simulink model "ForwardKinematic_YuMi"  (R2024a)
(part 9 of 23)

(5148155107303929*sin(q1L))/9007199254740992))/36893488147419103232 + sin(q2L)*((5148155107303929*cos(q1L))/9007199254740992 + (1888752292310023*sin(q1L))/18014398509481984)))/36893488147419103232 + cos(q3L)*((16506520352940097956833727997725*sin(q2L))/20282409603651670423947251286016 - cos(q2L)*((5148155107303929*cos(q1L))/9007199254740992 + (1888752292310023*sin(q1L))/18014398509481984) + (7514214926474921*sin(q2L)*((1888752292310023*cos(q1L))/18014398509481984 - (5148155107303929*sin(q1L))/9007199254740992))/36893488147419103232)))/332306998946228968225951765070086144 + (508577317689771495245073589786522929324694383585*sin(q3L)*((16506520352940097956833727997725*cos(q2L))/20282409603651670423947251286016 + (7514214926474921*cos(q2L)*((1888752292310023*cos(q1L))/18014398509481984 - (5148155107303929*sin(q1L))/9007199254740992))/36893488147419103232 + sin(q2L)*((5148155107303929*cos(q1L))/9007199254740992 + (1888752292310023*sin(q1L))/18014398509481984)))/12259964326927110866866776217202473468949912977468817408 - (67682029681889335677290557259385*cos(q3L)*((16506520352940097956833727997725*sin(q2L))/20282409603651670423947251286016 - cos(q2L)*((5148155107303929*cos(q1L))/9007199254740992 + (1888752292310023*sin(q1L))/18014398509481984) + (7514214926474921*sin(q2L)*((1888752292310023*cos(q1L))/18014398509481984 - (5148155107303929*sin(q1L))/9007199254740992))/36893488147419103232))/332306998946228968225951765070086144 + (1764482024691522628700660907665*sin(q3L)*((16506520352940097956833727997725*sin(q2L))/20282409603651670423947251286016 - cos(q2L)*((5148155107303929*cos(q1L))/9007199254740992 + (1888752292310023*sin(q1L))/18014398509481984) + (7514214926474921*sin(q2L)*((1888752292310023*cos(q1L))/18014398509481984 - (5148155107303929*sin(q1L))/9007199254740992))/36893488147419103232))/42535295865117307932921825928971026432))/16225927682921336339157801028812800 + (455490404115240510935077772268745492204390157443214084883134054419271951750419293234291596923751*cos(q3L)*((16506520352940097956833727997725*cos(q2L))/20282409603651670423947251286016 + (7514214926474921*cos(q2L)*((1888752292310023*cos(q1L))/18014398509481984 - (5148155107303929*sin(q1L))/9007199254740992))/36893488147419103232 + sin(q2L)*((5148155107303929*cos(q1L))/9007199254740992 + (1888752292310023*sin(q1L))/18014398509481984)))/53399675898022752059875542654238802865067613058916319248676040195555493144516013750574052173414400000 + (610321541873521657855151997354401418608858870661075444886782706002880706727*cos(q4L)*((9007199067919185*sin(q3L)*((46370457884011341126541404977865*sin(q1L))/81129638414606681695789005144064 - (17012367886825063216155529491255*cos(q1L))/162259276829213363391578010288128 + 13770489658876653055167369550485/83076749736557242056487941267521536))/9007199254740992 - (7514214926474921*sin(q3L)*((16506520352940097956833727997725*cos(q2L))/20282409603651670423947251286016 + (7514214926474921*cos(q2L)*((1888752292310023*cos(q1L))/18014398509481984 - (5148155107303929*sin(q1L))/9007199254740992))/36893488147419103232 + sin(q2L)*((5148155107303929*cos(q1L))/9007199254740992 + (1888752292310023*sin(q1L))/18014398509481984)))/36893488147419103232 + cos(q3L)*((16506520352940097956833727997725*sin(q2L))/20282409603651670423947251286016 - cos(q2L)*((5148155107303929*cos(q1L))/9007199254740992 + (1888752292310023*sin(q1L))/18014398509481984) + (7514214926474921*sin(q2L)*((1888752292310023*cos(q1L))/18014398509481984 - (5148155107303929*sin(q1L))/9007199254740992))/36893488147419103232)))/11307821214581659709333104004754678501295896940003961331978279688272766566400000 + (48638874966763599*sin(q6L)*((9007199067919185*((4503599440548691*cos(q4L))/4503599627370496 - (7514214926474921*sin(q4L))/36893488147419103232)*((7514214926474921*cos(q3L)*((16506520352940097956833727997725*cos(q2L))/20282409603651670423947251286016 + (7514214926474921*cos(q2L)*((1888752292310023*cos(q1L))/18014398509481984 - (5148155107303929*sin(q1L))/9007199254740992))/36893488147419103232 + sin(q2L)*((5148155107303929*cos(q1L))/9007199254740992 + (1888752292310023*sin(q1L))/18014398509481984)))/36893488147419103232 - (9007199067919185*cos(q3L)*((46370457884011341126541404977865*sin(q1L))/81129638414606681695789005144064 - (17012367886825063216155529491255*cos(q1L))/162259276829213363391578010288128 + 13770489658876653055167369550485/83076749736557242056487941267521536))/9007199254740992 + sin(q3L)*((16506520352940097956833727997725*sin(q2L))/20282409603651670423947251286016 - cos(q2L)*((5148155107303929*cos(q1L))/9007199254740992 + (1888752292310023*sin(q1L))/18014398509481984) + (7514214926474921*sin(q2L)*((1888752292310023*cos(q1L))/18014398509481984 - (5148155107303929*sin(q1L))/9007199254740992))/36893488147419103232)))/9007199254740992 - (609625514665592237562888769449172969868262801225*sin(q3L)*((46370457884011341126541404977865*sin(q1L))/81129638414606681695789005144064 - (17012367886825063216155529491255*cos(q1L))/162259276829213363391578010288128 + 13770489658876653055167369550485/83076749736557242056487941267521536))/2993155353253689176481146537402947624255349848014848 - (15893040848161638993908057577265778144967053025*cos(q3L)*((46370457884011341126541404977865*sin(q1L))/81129638414606681695789005144064 - (17012367886825063216155529491255*cos(q1L))/162259276829213363391578010288128 + 13770489658876653055167369550485/83076749736557242056487941267521536))/383123885216472214589586756787577295904684780545900544 + (13258697167433729449897784796786197386719169465*cos(q3L)*((16506520352940097956833727997725*cos(q2L))/20282409603651670423947251286016 + (7514214926474921*cos(q2L)*((1888752292310023*cos(q1L))/18014398509481984 - (5148155107303929*sin(q1L))/9007199254740992))/36893488147419103232 + sin(q2L)*((5148155107303929*cos(q1L))/9007199254740992 + (1888752292310023*sin(q1L))/18014398509481984)))/1569275433846670190958947355801916604025588861116008628224 + (67682029681889335677290557259385*cos(q4L)*((9007199067919185*sin(q3L)*((46370457884011341126541404977865*sin(q1L))/81129638414606681695789005144064 - (17012367886825063216155529491255*cos(q1L))/162259276829213363391578010288128 + 13770489658876653055167369550485/83076749736557242056487941267521536))/9007199254740992 - (7514214926474921*sin(q3L)*((16506520352940097956833727997725*cos(q2L))/20282409603651670423947251286016 + (7514214926474921*cos(q2L)*((1888752292310023*cos(q1L))/18014398509481984 - (5148155107303929*sin(q1L))/9007199254740992))/36893488147419103232 + sin(q2L)*((5148155107303929*cos(q1L))/9007199254740992 + (1888752292310023*sin(q1L))/18014398509481984)))/36893488147419103232 + cos(q3L)*((16506520352940097956833727997725*sin(q2L))/20282409603651670423947251286016 - cos(q2L)*((5148155107303929*cos(q1L))/9007199254740992 + (1888752292310023*sin(q1L))/18014398509481984) + (7514214926474921*sin(q2L)*((1888752292310023*cos(q1L))/18014398509481984 - (5148155107303929*sin(q1L))/9007199254740992))/36893488147419103232)))/332306998946228968225951765070086144 + (508577317689771495245073589786522929324694383585*sin(q3L)*((16506520352940097956833727997725*cos(q2L))/20282409603651670423947251286016 + (7514214926474921*cos(q2L)*((1888752292310023*cos(q1L))/18014398509481984 - (5148155107303929*sin(q1L))/9007199254740992))/36893488147419103232 + sin(q2L)*((5148155107303929*cos(q1L))/9007199254740992 + (1888752292310023*sin(q1L))/18014398509481984)))/12259964326927110866866776217202473468949912977468817408 - (67682029681889335677290557259385*cos(q3L)*((16506520352940097956833727997725*sin(q2L))/20282409603651670423947251286016 - cos(q2L)*((5148155107303929*cos(q1L))/9007199254740992 + (1888752292310023*sin(q1L))/18014398509481984) + (7514214926474921*sin(q2L)*((1888752292310023*cos(q1L))/18014398509481984 - (5148155107303929*sin(q1L))/9007199254740992))/36893488147419103232))/332306998946228968225951765070086144 + (1764482024691522628700660907665*sin(q3L)*((16506520352940097956833727997725*sin(q2L))/20282409603651670423947251286016 - cos(q2L)*((5148155107303929*cos(q1L))/9007199254740992 + (1888752292310023*sin(q1L))/18014398509481984) + (7514214926474921*sin(q2L)*((1888752292310023*cos(q1L))/18014398509481984 - (5148155107303929*sin(q1L))/9007199254740992))/36893488147419103232))/42535295865117307932921825928971026432))/1801439850948198400 + (2436553109258773196144549622003023*cos(q6L)*((7514214926474921*cos(q5L)*(((4503599440548691*cos(q4L))/4503599627370496 - (7514214926474921*sin(q4L))/36893488147419103232)*((7514214926474921*cos(q3L)*((16506520352940097956833727997725*cos(q2L))/20282409603651670423947251286016 + (7514214926474921*cos(q2L)*((1888752292310023*cos(q1L))/18014398509481984 - (5148155107303929*sin(q1L))/9007199254740992))/36893488147419103232 + sin(q2L)*((5148155107303929*cos(q1L))/9007199254740992 + (1888752292310023*sin(q1L))/18014398509481984)))/36893488147419103232 - (9007199067919185*cos(q3L)*((46370457884011341126541404977865*sin(q1L))/81129638414606681695789005144064 - (17012367886825063216155529491255*cos(q1L))/162259276829213363391578010288128 + 13770489658876653055167369550485/83076749736557242056487941267521536))/9007199254740992 + sin(q3L)*((16506520352940097956833727997725*sin(q2L))/20282409603651670423947251286016 - cos(q2L)*((5148155107303929*cos(q1L))/9007199254740992 + (1888752292310023*sin(q1L))/18014398509481984) + (7514214926474921*sin(q2L)*((1888752292310023*cos(q1L))/18014398509481984 - (5148155107303929*sin(q1L))/9007199254740992))/36893488147419103232)) + (7514214926474921*cos(q4L)*((9007199067919185*sin(q3L)*((46370457884011341126541404977865*sin(q1L))/81129638414606681695789005144064 - (17012367886825063216155529491255*cos(q1L))/162259276829213363391578010288128 + 13770489658876653055167369550485/83076749736557242056487941267521536))/9007199254740992 - (7514214926474921*sin(q3L)*((16506520352940097956833727997725*cos(q2L))/20282409603651670423947251286016 + (7514214926474921*cos(q2L)*((1888752292310023*cos(q1L))/18014398509481984 - (5148155107303929*sin(q1L))/9007199254740992))/36893488147419103232 + sin(q2L)*((5148155107303929*cos(q1L))/9007199254740992 + (1888752292310023*sin(q1L))/18014398509481984)))/36893488147419103232 + cos(q3L)*((16506520352940097956833727997725*sin(q2L))/20282409603651670423947251286016 - cos(q2L)*((5148155107303929*cos(q1L))/9007199254740992 + (1888752292310023*sin(q1L))/18014398509481984) + (7514214926474921*sin(q2L)*((1888752292310023*cos(q1L))/18014398509481984 - (5148155107303929*sin(q1L))/9007199254740992))/36893488147419103232)))/36893488147419103232))/36893488147419103232 + sin(q5L)*(((7514214926474921*cos(q4L))/36893488147419103232 + (4503599440548691*sin(q4L))/4503599627370496)*((7514214926474921*cos(q3L)*((16506520352940097956833727997725*cos(q2L))/20282409603651670423947251286016 + (7514214926474921*cos(q2L)*((1888752292310023*cos(q1L))/18014398509481984 - (5148155107303929*sin(q1L))/9007199254740992))/36893488147419103232 + sin(q2L)*((5148155107303929*cos(q1L))/9007199254740992 + (1888752292310023*sin(q1L))/18014398509481984)))/36893488147419103232 - (9007199067919185*cos(q3L)*((46370457884011341126541404977865*sin(q1L))/81129638414606681695789005144064 - (17012367886825063216155529491255*cos(q1L))/162259276829213363391578010288128 + 13770489658876653055167369550485/83076749736557242056487941267521536))/9007199254740992 + sin(q3L)*((16506520352940097956833727997725*sin(q2L))/20282409603651670423947251286016 - cos(q2L)*((5148155107303929*cos(q1L))/9007199254740992 + (1888752292310023*sin(q1L))/18014398509481984) + (7514214926474921*sin(q2L)*((1888752292310023*cos(q1L))/18014398509481984 - (5148155107303929*sin(q1L))/9007199254740992))/36893488147419103232)) + (7514214926474921*sin(q4L)*((9007199067919185*sin(q3L)*((46370457884011341126541404977865*sin(q1L))/81129638414606681695789005144064 - (17012367886825063216155529491255*cos(q1L))/162259276829213363391578010288128 + 13770489658876653055167369550485/83076749736557242056487941267521536))/9007199254740992 - (7514214926474921*sin(q3L)*((16506520352940097956833727997725*cos(q2L))/20282409603651670423947251286016 + (7514214926474921*cos(q2L)*((1888752292310023*cos(q1L))/18014398509481984 - (5148155107303929*sin(q1L))/9007199254740992))/36893488147419103232 + sin(q2L)*((5148155107303929*cos(q1L))/9007199254740992 + (1888752292310023*sin(q1L))/18014398509481984)))/36893488147419103232 + cos(q3L)*((16506520352940097956833727997725*sin(q2L))/20282409603651670423947251286016 - cos(q2L)*((5148155107303929*cos(q1L))/9007199254740992 + (1888752292310023*sin(q1L))/18014398509481984) + (7514214926474921*sin(q2L)*((1888752292310023*cos(q1L))/18014398509481984 - (5148155107303929*sin(q1L))/9007199254740992))/36893488147419103232)))/36893488147419103232) + (9007199067919185*cos(q5L)*((2115063383689692319117831580025*cos(q3L)*((46370457884011341126541404977865*sin(q1L))/81129638414606681695789005144064 - (17012367886825063216155529491255*cos(q1L))/162259276829213363391578010288128 + 13770489658876653055167369550485/83076749736557242056487941267521536))/10384593717069655257060992658440192 + (81129635049124235038645691064225*sin(q3L)*((46370457884011341126541404977865*sin(q1L))/81129638414606681695789005144064 - (17012367886825063216155529491255*cos(q1L))/162259276829213363391578010288128 + 13770489658876653055167369550485/83076749736557242056487941267521536))/81129638414606681695789005144064 - (1764482024691522628700660907665*cos(q3L)*((16506520352940097956833727997725*cos(q2L))/20282409603651670423947251286016 + (7514214926474921*cos(q2L)*((1888752292310023*cos(q1L))/18014398509481984 - (5148155107303929*sin(q1L))/9007199254740992))/36893488147419103232 + sin(q2L)*((5148155107303929*cos(q1L))/9007199254740992 + (1888752292310023*sin(q1L))/18014398509481984)))/42535295865117307932921825928971026432 - (67682029681889335677290557259385*sin(q3L)*((16506520352940097956833727997725*cos(q2L))/20282409603651670423947251286016 + (7514214926474921*cos(q2L)*((1888752292310023*cos(q1L))/18014398509481984 - (5148155107303929*sin(q1L))/9007199254740992))/36893488147419103232 + sin(q2L)*((5148155107303929*cos(q1L))/9007199254740992 + (1888752292310023*sin(q1L))/18014398509481984)))/332306998946228968225951765070086144 + (9007199067919185*cos(q3L)*((16506520352940097956833727997725*sin(q2L))/20282409603651670423947251286016 - cos(q2L)*((5148155107303929*cos(q1L))/9007199254740992 + (1888752292310023*sin(q1L))/18014398509481984) + (7514214926474921*sin(q2L)*((1888752292310023*cos(q1L))/18014398509481984 - (5148155107303929*sin(q1L))/9007199254740992))/36893488147419103232))/9007199254740992 - (234819211581865*sin(q3L)*((16506520352940097956833727997725*sin(q2L))/20282409603651670423947251286016 - cos(q2L)*((5148155107303929*cos(q1L))/9007199254740992 + (1888752292310023*sin(q1L))/18014398509481984) + (7514214926474921*sin(q2L)*((1888752292310023*cos(q1L))/18014398509481984 - (5148155107303929*sin(q1L))/9007199254740992))/36893488147419103232))/1152921504606846976))/9007199254740992))/332306998946228968225951765070086144000 + (347469655025336708709976918716104493695816557877713443586884917071777956519687017125887603*sin(q3L)*((16506520352940097956833727997725*cos(q2L))/20282409603651670423947251286016 + (7514214926474921*cos(q2L)*((1888752292310023*cos(q1L))/18014398509481984 - (5148155107303929*sin(q1L))/9007199254740992))/36893488147419103232 + sin(q2L)*((5148155107303929*cos(q1L))/9007199254740992 + (1888752292310023*sin(q1L))/18014398509481984)))/83436993590660550093555535397248129476668145404556748826056312805555458038306271485271956520960000 - (46241644459901303158631016767207157814229090534989303509431886332469146043*cos(q3L)*((16506520352940097956833727997725*sin(q2L))/20282409603651670423947251286016 - cos(q2L)*((5148155107303929*cos(q1L))/9007199254740992 + (1888752292310023*sin(q1L))/18014398509481984) + (7514214926474921*sin(q2L)*((1888752292310023*cos(q1L))/18014398509481984 - (5148155107303929*sin(q1L))/9007199254740992))/36893488147419103232))/2261564242916331941866620800950935700259179388000792266395655937654553313280000 + (608651409044468601*sin(q4L)*((9007199067919185*sin(q3L)*((46370457884011341126541404977865*sin(q1L))/81129638414606681695789005144064 - (17012367886825063216155529491255*cos(q1L))/162259276829213363391578010288128 + 13770489658876653055167369550485/83076749736557242056487941267521536))/9007199254740992 - (7514214926474921*sin(q3L)*((16506520352940097956833727997725*cos(q2L))/20282409603651670423947251286016 + (7514214926474921*cos(q2L)*((1888752292310023*cos(q1L))/18014398509481984 - (5148155107303929*sin(q1L))/9007199254740992))/36893488147419103232 + sin(q2L)*((5148155107303929*cos(q1L))/9007199254740992 + (1888752292310023*sin(q1L))/18014398509481984)))/36893488147419103232 + cos(q3L)*((16506520352940097956833727997725*sin(q2L))/20282409603651670423947251286016 - cos(q2L)*((5148155107303929*cos(q1L))/9007199254740992 + (1888752292310023*sin(q1L))/18014398509481984) + (7514214926474921*sin(q2L)*((1888752292310023*cos(q1L))/18014398509481984 - (5148155107303929*sin(q1L))/9007199254740992))/36893488147419103232)))/73786976294838206464000 + (202883803014822867*sin(q6L)*((7514214926474921*cos(q5L)*(((4503599440548691*cos(q4L))/4503599627370496 - (7514214926474921*sin(q4L))/36893488147419103232)*((7514214926474921*cos(q3L)*((16506520352940097956833727997725*cos(q2L))/20282409603651670423947251286016 + (7514214926474921*cos(q2L)*((1888752292310023*cos(q1L))/18014398509481984 - (5148155107303929*sin(q1L))/9007199254740992))/36893488147419103232 + sin(q2L)*((5148155107303929*cos(q1L))/9007199254740992 + (1888752292310023*sin(q1L))/18014398509481984)))/36893488147419103232 - (9007199067919185*cos(q3L)*((46370457884011341126541404977865*sin(q1L))/81129638414606681695789005144064 - (17012367886825063216155529491255*cos(q1L))/162259276829213363391578010288128 + 13770489658876653055167369550485/83076749736557242056487941267521536))/9007199254740992 + sin(q3L)*((16506520352940097956833727997725*sin(q2L))/20282409603651670423947251286016 - cos(q2L)*((5148155107303929*cos(q1L))/9007199254740992 + (1888752292310023*sin(q1L))/18014398509481984) + (7514214926474921*sin(q2L)*((1888752292310023*cos(q1L))/18014398509481984 - (5148155107303929*sin(q1L))/9007199254740992))/36893488147419103232)) + (7514214926474921*cos(q4L)*((9007199067919185*sin(q3L)*((46370457884011341126541404977865*sin(q1L))/81129638414606681695789005144064 - (17012367886825063216155529491255*cos(q1L))/162259276829213363391578010288128 + 13770489658876653055167369550485/83076749736557242056487941267521536))/9007199254740992 - (7514214926474921*sin(q3L)*((16506520352940097956833727997725*cos(q2L))/20282409603651670423947251286016 + (7514214926474921*cos(q2L)*((1888752292310023*cos(q1L))/18014398509481984 - (5148155107303929*sin(q1L))/9007199254740992))/36893488147419103232 + sin(q2L)*((5148155107303929*cos(q1L))/9007199254740992 + (1888752292310023*sin(q1L))/18014398509481984)))/36893488147419103232 + cos(q3L)*((16506520352940097956833727997725*sin(q2L))/20282409603651670423947251286016 - cos(q2L)*((5148155107303929*cos(q1L))/9007199254740992 + (1888752292310023*sin(q1L))/18014398509481984) + (7514214926474921*sin(q2L)*((1888752292310023*cos(q1L))/18014398509481984 - (5148155107303929*sin(q1L))/9007199254740992))/36893488147419103232)))/36893488147419103232))/36893488147419103232 + sin(q5L)*(((7514214926474921*cos(q4L))/36893488147419103232 + (4503599440548691*sin(q4L))/4503599627370496)*((7514214926474921*cos(q3L)*((16506520352940097956833727997725*cos(q2L))/20282409603651670423947251286016 + (7514214926474921*cos(q2L)*((1888752292310023*cos(q1L))/18014398509481984 - (5148155107303929*sin(q1L))/9007199254740992))/36893488147419103232 + sin(q2L)*((5148155107303929*cos(q1L))/9007199254740992 + (1888752292310023*sin(q1L))/18014398509481984)))/36893488147419103232 - (9007199067919185*cos(q3L)*((46370457884011341126541404977865*sin(q1L))/81129638414606681695789005144064 - (17012367886825063216155529491255*cos(q1L))/162259276829213363391578010288128 + 13770489658876653055167369550485/83076749736557242056487941267521536))/9007199254740992 + sin(q3L)*((16506520352940097956833727997725*sin(q2L))/20282409603651670423947251286016 - cos(q2L)*((5148155107303929*cos(q1L))/9007199254740992 + (1888752292310023*sin(q1L))/18014398509481984) + (7514214926474921*sin(q2L)*((1888752292310023*cos(q1L))/18014398509481984 - (5148155107303929*sin(q1L))/9007199254740992))/36893488147419103232)) + (7514214926474921*sin(q4L)*((9007199067919185*sin(q3L)*((46370457884011341126541404977865*sin(q1L))/81129638414606681695789005144064 - (17012367886825063216155529491255*cos(q1L))/162259276829213363391578010288128 + 13770489658876653055167369550485/83076749736557242056487941267521536))/9007199254740992 - (7514214926474921*sin(q3L)*((16506520352940097956833727997725*cos(q2L))/20282409603651670423947251286016 + (7514214926474921*cos(q2L)*((1888752292310023*cos(q1L))/18014398509481984 - (5148155107303929*sin(q1L))/9007199254740992))/36893488147419103232 + sin(q2L)*((5148155107303929*cos(q1L))/9007199254740992 + (1888752292310023*sin(q1L))/18014398509481984)))/36893488147419103232 + cos(q3L)*((16506520352940097956833727997725*sin(q2L))/20282409603651670423947251286016 - cos(q2L)*((5148155107303929*cos(q1L))/9007199254740992 + (1888752292310023*sin(q1L))/18014398509481984) + (7514214926474921*sin(q2L)*((1888752292310023*cos(q1L))/18014398509481984 - (5148155107303929*sin(q1L))/9007199254740992))/36893488147419103232)))/36893488147419103232) + (9007199067919185*cos(q5L)*((2115063383689692319117831580025*cos(q3L)*((46370457884011341126541404977865*sin(q1L))/81129638414606681695789005144064 - (17012367886825063216155529491255*cos(q1L))/162259276829213363391578010288128 + 13770489658876653055167369550485/83076749736557242056487941267521536))/10384593717069655257060992658440192 + (81129635049124235038645691064225*sin(q3L)*((46370457884011341126541404977865*sin(q1L))/81129638414606681695789005144064 - (17012367886825063216155529491255*cos(q1L))/162259276829213363391578010288128 + 13770489658876653055167369550485/83076749736557242056487941267521536))/81129638414606681695789005144064 - (1764482024691522628700660907665*cos(q3L)*((16506520352940097956833727997725*cos(q2L))/20282409603651670423947251286016 + (7514214926474921*cos(q2L)*((1888752292310023*cos(q1L))/18014398509481984 - (5148155107303929*sin(q1L))/9007199254740992))/36893488147419103232 + sin(q2L)*((5148155107303929*cos(q1L))/9007199254740992 + (1888752292310023*sin(q1L))/18014398509481984)))/42535295865117307932921825928971026432 - (67682029681889335677290557259385*sin(q3L)*((16506520352940097956833727997725*cos(q2L))/20282409603651670423947251286016 + (7514214926474921*cos(q2L)*((1888752292310023*cos(q1L))/18014398509481984 - (5148155107303929*sin(q1L))/9007199254740992))/36893488147419103232 + sin(q2L)*((5148155107303929*cos(q1L))/9007199254740992 + (1888752292310023*sin(q1L))/18014398509481984)))/332306998946228968225951765070086144 + (9007199067919185*cos(q3L)*((16506520352940097956833727997725*sin(q2L))/20282409603651670423947251286016 - cos(q2L)*((5148155107303929*cos(q1L))/9007199254740992 + (1888752292310023*sin(q1L))/18014398509481984) + (7514214926474921*sin(q2L)*((1888752292310023*cos(q1L))/18014398509481984 - (5148155107303929*sin(q1L))/9007199254740992))/36893488147419103232))/9007199254740992 - (234819211581865*sin(q3L)*((16506520352940097956833727997725*sin(q2L))/20282409603651670423947251286016 - cos(q2L)*((5148155107303929*cos(q1L))/9007199254740992 + (1888752292310023*sin(q1L))/18014398509481984) + (7514214926474921*sin(q2L)*((1888752292310023*cos(q1L))/18014398509481984 - (5148155107303929*sin(q1L))/9007199254740992))/36893488147419103232))/1152921504606846976))/9007199254740992))/36893488147419103232000 - (27*cos(q6L)*((7514214926474921*sin(q5L)*(((4503599440548691*cos(q4L))/4503599627370496 - (7514214926474921*sin(q4L))/36893488147419103232)*((7514214926474921*cos(q3L)*((16506520352940097956833727997725*cos(q2L))/20282409603651670423947251286016 + (7514214926474921*cos(q2L)*((1888752292310023*cos(q1L))/18014398509481984 - (5148155107303929*sin(q1L))/9007199254740992))/36893488147419103232 + sin(q2L)*((5148155107303929*cos(q1L))/9007199254740992 + (1888752292310023*sin(q1L))/18014398509481984)))/36893488147419103232 - (9007199067919185*cos(q3L)*((46370457884011341126541404977865*sin(q1L))/81129638414606681695789005144064 - (17012367886825063216155529491255*cos(q1L))/162259276829213363391578010288128 + 13770489658876653055167369550485/83076749736557242056487941267521536))/9007199254740992 + sin(q3L)*((16506520352940097956833727997725*sin(q2L))/20282409603651670423947251286016 - cos(q2L)*((5148155107303929*cos(q1L))/9007199254740992 + (1888752292310023*sin(q1L))/18014398509481984) + (7514214926474921*sin(q2L)*((1888752292310023*cos(q1L))/18014398509481984 - (5148155107303929*sin(q1L))/9007199254740992))/36893488147419103232)) + (7514214926474921*cos(q4L)*((9007199067919185*sin(q3L)*((46370457884011341126541404977865*sin(q1L))/81129638414606681695789005144064 - (17012367886825063216155529491255*cos(q1L))/162259276829213363391578010288128 + 13770489658876653055167369550485/83076749736557242056487941267521536))/9007199254740992 - (7514214926474921*sin(q3L)*((16506520352940097956833727997725*cos(q2L))/20282409603651670423947251286016 + (7514214926474921*cos(q2L)*((1888752292310023*cos(q1L))/18014398509481984 - (5148155107303929*sin(q1L))/9007199254740992))/36893488147419103232 + sin(q2L)*((5148155107303929*cos(q1L))/9007199254740992 + (1888752292310023*sin(q1L))/18014398509481984)))/36893488147419103232 + cos(q3L)*((16506520352940097956833727997725*sin(q2L))/20282409603651670423947251286016 - cos(q2L)*((5148155107303929*cos(q1L))/9007199254740992 + (1888752292310023*sin(q1L))/18014398509481984) + (7514214926474921*sin(q2L)*((1888752292310023*cos(q1L))/18014398509481984 - (5148155107303929*sin(q1L))/9007199254740992))/36893488147419103232)))/36893488147419103232))/36893488147419103232 - cos(q5L)*(((7514214926474921*cos(q4L))/36893488147419103232 + (4503599440548691*sin(q4L))/4503599627370496)*((7514214926474921*cos(q3L)*((16506520352940097956833727997725*cos(q2L))/20282409603651670423947251286016 + (7514214926474921*cos(q2L)*((1888752292310023*cos(q1L))/18014398509481984 - (5148155107303929*sin(q1L))/9007199254740992))/36893488147419103232 + sin(q2L)*((5148155107303929*cos(q1L))/9007199254740992 + (1888752292310023*sin(q1L))/18014398509481984)))/36893488147419103232 - (9007199067919185*cos(q3L)*((46370457884011341126541404977865*sin(q1L))/81129638414606681695789005144064 - (17012367886825063216155529491255*cos(q1L))/162259276829213363391578010288128 + 13770489658876653055167369550485/83076749736557242056487941267521536))/9007199254740992 + sin(q3L)*((16506520352940097956833727997725*sin(q2L))/20282409603651670423947251286016 - cos(q2L)*((5148155107303929*cos(q1L))/9007199254740992 + (1888752292310023*sin(q1L))/18014398509481984) + (7514214926474921*sin(q2L)*((1888752292310023*cos(q1L))/18014398509481984 - (5148155107303929*sin(q1L))/9007199254740992))/36893488147419103232)) + (7514214926474921*sin(q4L)*((9007199067919185*sin(q3L)*((46370457884011341126541404977865*sin(q1L))/81129638414606681695789005144064 - (17012367886825063216155529491255*cos(q1L))/162259276829213363391578010288128 + 13770489658876653055167369550485/83076749736557242056487941267521536))/9007199254740992 - (7514214926474921*sin(q3L)*((16506520352940097956833727997725*cos(q2L))/20282409603651670423947251286016 + (7514214926474921*cos(q2L)*((1888752292310023*cos(q1L))/18014398509481984 - (5148155107303929*sin(q1L))/9007199254740992))/36893488147419103232 + sin(q2L)*((5148155107303929*cos(q1L))/9007199254740992 + (1888752292310023*sin(q1L))/18014398509481984)))/36893488147419103232 + cos(q3L)*((16506520352940097956833727997725*sin(q2L))/20282409603651670423947251286016 - cos(q2L)*((5148155107303929*cos(q1L))/9007199254740992 + (1888752292310023*sin(q1L))/18014398509481984) + (7514214926474921*sin(q2L)*((1888752292310023*cos(q1L))/18014398509481984 - (5148155107303929*sin(q1L))/9007199254740992))/36893488147419103232)))/36893488147419103232) + (9007199067919185*sin(q5L)*((2115063383689692319117831580025*cos(q3L)*((46370457884011341126541404977865*sin(q1L))/81129638414606681695789005144064 - (17012367886825063216155529491255*cos(q1L))/162259276829213363391578010288128 + 13770489658876653055167369550485/83076749736557242056487941267521536))/10384593717069655257060992658440192 + (81129635049124235038645691064225*sin(q3L)*((46370457884011341126541404977865*sin(q1L))/81129638414606681695789005144064 - (17012367886825063216155529491255*cos(q1L))/162259276829213363391578010288128 + 13770489658876653055167369550485/83076749736557242056487941267521536))/81129638414606681695789005144064 - (1764482024691522628700660907665*cos(q3L)*((16506520352940097956833727997725*cos(q2L))/20282409603651670423947251286016 + (7514214926474921*cos(q2L)*((1888752292310023*cos(q1L))/18014398509481984 - (5148155107303929*sin(q1L))/9007199254740992))/36893488147419103232 + sin(q2L)*((5148155107303929*cos(q1L))/9007199254740992 + (1888752292310023*sin(q1L))/18014398509481984)))/42535295865117307932921825928971026432 - (67682029681889335677290557259385*sin(q3L)*((16506520352940097956833727997725*cos(q2L))/20282409603651670423947251286016 + (7514214926474921*cos(q2L)*((1888752292310023*cos(q1L))/18014398509481984 - (5148155107303929*sin(q1L))/9007199254740992))/36893488147419103232 + sin(q2L)*((5148155107303929*cos(q1L))/9007199254740992 + (1888752292310023*sin(q1L))/18014398509481984)))/332306998946228968225951765070086144 + (9007199067919185*cos(q3L)*((16506520352940097956833727997725*sin(q2L))/20282409603651670423947251286016 - cos(q2L)*((5148155107303929*cos(q1L))/9007199254740992 + (1888752292310023*sin(q1L))/18014398509481984) + (7514214926474921*sin(q2L)*((1888752292310023*cos(q1L))/18014398509481984 - (5148155107303929*sin(q1L))/9007199254740992))/36893488147419103232))/9007199254740992 - (234819211581865*sin(q3L)*((16506520352940097956833727997725*sin(q2L))/20282409603651670423947251286016 - cos(q2L)*((5148155107303929*cos(q1L))/9007199254740992 + (1888752292310023*sin(q1L))/18014398509481984) + (7514214926474921*sin(q2L)*((1888752292310023*cos(q1L))/18014398509481984 - (5148155107303929*sin(q1L))/9007199254740992))/36893488147419103232))/1152921504606846976))/9007199254740992))/1000 + (60617164743372705924380750591060836759586313939367162716784907429017787816377231*sin(q3L)*((16506520352940097956833727997725*sin(q2L))/20282409603651670423947251286016 - cos(q2L)*((5148155107303929*cos(q1L))/9007199254740992 + (1888752292310023*sin(q1L))/18014398509481984) + (7514214926474921*sin(q2L)*((1888752292310023*cos(q1L))/18014398509481984 - (5148155107303929*sin(q1L))/9007199254740992))/36893488147419103232))/1447401115466452442794637312608598848165874808320507050493219800098914120499200000 + (324259171862923063*sin(q6L)*((7514214926474921*sin(q5L)*(((4503599440548691*cos(q4L))/4503599627370496 - (7514214926474921*sin(q4L))/36893488147419103232)*((7514214926474921*cos(q3L)*((16506520352940097956833727997725*cos(q2L))/20282409603651670423947251286016 + (7514214926474921*cos(q2L)*((1888752292310023*cos(q1L))/18014398509481984 - (5148155107303929*sin(q1L))/9007199254740992))/36893488147419103232 + sin(q2L)*((5148155107303929*cos(q1L))/9007199254740992 + (1888752292310023*sin(q1L))/18014398509481984)))/36893488147419103232 - (9007199067919185*cos(q3L)*((46370457884011341126541404977865*sin(q1L))/81129638414606681695789005144064 - (17012367886825063216155529491255*cos(q1L))/162259276829213363391578010288128 + 13770489658876653055167369550485/83076749736557242056487941267521536))/9007199254740992 + sin(q3L)*((16506520352940097956833727997725*sin(q2L))/20282409603651670423947251286016 - cos(q2L)*((5148155107303929*cos(q1L))/9007199254740992 + (1888752292310023*sin(q1L))/18014398509481984) + (7514214926474921*sin(q2L)*((1888752292310023*cos(q1L))/18014398509481984 - (5148155107303929*sin(q1L))/9007199254740992))/36893488147419103232)) + (7514214926474921*cos(q4L)*((9007199067919185*sin(q3L)*((46370457884011341126541404977865*sin(q1L))/81129638414606681695789005144064 - (17012367886825063216155529491255*cos(q1L))/162259276829213363391578010288128 + 13770489658876653055167369550485/83076749736557242056487941267521536))/9007199254740992 - (7514214926474921*sin(q3L)*((16506520352940097956833727997725*cos(q2L))/20282409603651670423947251286016 + (7514214926474921*cos(q2L)*((1888752292310023*cos(q1L))/18014398509481984 - (5148155107303929*sin(q1L))/9007199254740992))/36893488147419103232 + sin(q2L)*((5148155107303929*cos(q1L))/9007199254740992 + (1888752292310023*sin(q1L))/18014398509481984)))/36893488147419103232 + cos(q3L)*((16506520352940097956833727997725*sin(q2L))/20282409603651670423947251286016 - cos(q2L)*((5148155107303929*cos(q1L))/9007199254740992 + (1888752292310023*sin(q1L))/18014398509481984) + (7514214926474921*sin(q2L)*((1888752292310023*cos(q1L))/18014398509481984 - (5148155107303929*sin(q1L))/9007199254740992))/36893488147419103232)))/36893488147419103232))/36893488147419103232 - cos(q5L)*(((7514214926474921*cos(q4L))/36893488147419103232 + (4503599440548691*sin(q4L))/4503599627370496)*((7514214926474921*cos(q3L)*((16506520352940097956833727997725*cos(q2L))/20282409603651670423947251286016 + (7514214926474921*cos(q2L)*((1888752292310023*cos(q1L))/18014398509481984 - (5148155107303929*sin(q1L))/9007199254740992))/36893488147419103232 + sin(q2L)*((5148155107303929*cos(q1L))/9007199254740992 + (1888752292310023*sin(q1L))/18014398509481984)))/36893488147419103232 - (9007199067919185*cos(q3L)*((46370457884011341126541404977865*sin(q1L))/81129638414606681695789005144064 - (17012367886825063216155529491255*cos(q1L))/162259276829213363391578010288128 + 13770489658876653055167369550485/83076749736557242056487941267521536))/9007199254740992 + sin(q3L)*((16506520352940097956833727997725*sin(q2L))/20282409603651670423947251286016 - cos(q2L)*((5148155107303929*cos(q1L))/9007199254740992 + (1888752292310023*sin(q1L))/18014398509481984) + (7514214926474921*sin(q2L)*((1888752292310023*cos(q1L))/18014398509481984 - (5148155107303929*sin(q1L))/9007199254740992))/36893488147419103232)) + (7514214926474921*sin(q4L)*((9007199067919185*sin(q3L)*((46370457884011341126541404977865*sin(q1L))/81129638414606681695789005144064 - (17012367886825063216155529491255*cos(q1L))/162259276829213363391578010288128 + 13770489658876653055167369550485/83076749736557242056487941267521536))/9007199254740992 - (7514214926474921*sin(q3L)*((16506520352940097956833727997725*cos(q2L))/20282409603651670423947251286016 + (7514214926474921*cos(q2L)*((1888752292310023*cos(q1L))/18014398509481984 - (5148155107303929*sin(q1L))/9007199254740992))/36893488147419103232 + sin(q2L)*((5148155107303929*cos(q1L))/9007199254740992 + (1888752292310023*sin(q1L))/18014398509481984)))/36893488147419103232 + cos(q3L)*((16506520352940097956833727997725*sin(q2L))/20282409603651670423947251286016 - cos(q2L)*((5148155107303929*cos(q1L))/9007199254740992 + (1888752292310023*sin(q1L))/18014398509481984) + (7514214926474921*sin(q2L)*((1888752292310023*cos(q1L))/18014398509481984 - (5148155107303929*sin(q1L))/9007199254740992))/36893488147419103232)))/36893488147419103232) + (9007199067919185*sin(q5L)*((2115063383689692319117831580025*cos(q3L)*((46370457884011341126541404977865*sin(q1L))/81129638414606681695789005144064 - (17012367886825063216155529491255*cos(q1L))/162259276829213363391578010288128 + 13770489658876653055167369550485/83076749736557242056487941267521536))/10384593717069655257060992658440192 + (81129635049124235038645691064225*sin(q3L)*((46370457884011341126541404977865*sin(q1L))/81129638414606681695789005144064 - (17012367886825063216155529491255*cos(q1L))/162259276829213363391578010288128 + 13770489658876653055167369550485/83076749736557242056487941267521536))/81129638414606681695789005144064 - (1764482024691522628700660907665*cos(q3L)*((16506520352940097956833727997725*cos(q2L))/20282409603651670423947251286016 + (7514214926474921*cos(q2L)*((1888752292310023*cos(q1L))/18014398509481984 - (5148155107303929*sin(q1L))/9007199254740992))/36893488147419103232 + sin(q2L)*((5148155107303929*cos(q1L))/9007199254740992 + (1888752292310023*sin(q1L))/18014398509481984)))/42535295865117307932921825928971026432 - (67682029681889335677290557259385*sin(q3L)*((16506520352940097956833727997725*cos(q2L))/20282409603651670423947251286016 + (7514214926474921*cos(q2L)*((1888752292310023*cos(q1L))/18014398509481984 - (5148155107303929*sin(q1L))/9007199254740992))/36893488147419103232 + sin(q2L)*((5148155107303929*cos(q1L))/9007199254740992 + (1888752292310023*sin(q1L))/18014398509481984)))/332306998946228968225951765070086144 + (9007199067919185*cos(q3L)*((16506520352940097956833727997725*sin(q2L))/20282409603651670423947251286016 - cos(q2L)*((5148155107303929*cos(q1L))/9007199254740992 + (1888752292310023*sin(q1L))/18014398509481984) + (7514214926474921*sin(q2L)*((1888752292310023*cos(q1L))/18014398509481984 - (5148155107303929*sin(q1L))/9007199254740992))/36893488147419103232))/9007199254740992 - (234819211581865*sin(q3L)*((16506520352940097956833727997725*sin(q2L))/20282409603651670423947251286016 - cos(q2L)*((5148155107303929*cos(q1L))/9007199254740992 + (1888752292310023*sin(q1L))/18014398509481984) + (7514214926474921*sin(q2L)*((1888752292310023*cos(q1L))/18014398509481984 - (5148155107303929*sin(q1L))/9007199254740992))/36893488147419103232))/1152921504606846976))/9007199254740992))/9007199254740992000, (81222263116692158804177042061221826384594597321566869716687*((7514214926474921*cos(q4L))/36893488147419103232 + (4503599440548691*sin(q4L))/4503599627370496)*((9007199067919185*sin(q3L)*((46370457884011341126541404977865*sin(q1L))/81129638414606681695789005144064 - (17012367886825063216155529491255*cos(q1L))/162259276829213363391578010288128 + 13770489658876653055167369550485/83076749736557242056487941267521536))/9007199254740992 - (7514214926474921*sin(q3L)*((16506520352940097956833727997725*cos(q2L))/20282409603651670423947251286016 + (7514214926474921*cos(q2L)*((1888752292310023*cos(q1L))/18014398509481984 - (5148155107303929*sin(q1L))/9007199254740992))/36893488147419103232 + sin(q2L)*((5148155107303929*cos(q1L))/9007199254740992 + (1888752292310023*sin(q1L))/18014398509481984)))/36893488147419103232 + cos(q3L)*((16506520352940097956833727997725*sin(q2L))/20282409603651670423947251286016 - cos(q2L)*((5148155107303929*cos(q1L))/9007199254740992 + (1888752292310023*sin(q1L))/18014398509481984) + (7514214926474921*sin(q2L)*((1888752292310023*cos(q1L))/18014398509481984 - (5148155107303929*sin(q1L))/9007199254740992))/36893488147419103232)))/306499108173177771671669405430061836723747824436720435200000 - (81*((4503599440548691*cos(q4L))/4503599627370496 - (7514214926474921*sin(q4L))/36893488147419103232)*((9007199067919185*sin(q3L)*((46370457884011341126541404977865*sin(q1L))/81129638414606681695789005144064 - (17012367886825063216155529491255*cos(q1L))/162259276829213363391578010288128 + 13770489658876653055167369550485/83076749736557242056487941267521536))/9007199254740992 - (7514214926474921*sin(q3L)*((16506520352940097956833727997725*cos(q2L))/20282409603651670423947251286016 + (7514214926474921*cos(q2L)*((1888752292310023*cos(q1L))/18014398509481984 - (5148155107303929*sin(q1L))/9007199254740992))/36893488147419103232 + sin(q2L)*((5148155107303929*cos(q1L))/9007199254740992 + (1888752292310023*sin(q1L))/18014398509481984)))/36893488147419103232 + cos(q3L)*((16506520352940097956833727997725*sin(q2L))/20282409603651670423947251286016 - cos(q2L)*((5148155107303929*cos(q1L))/9007199254740992 + (1888752292310023*sin(q1L))/18014398509481984) + (7514214926474921*sin(q2L)*((1888752292310023*cos(q1L))/18014398509481984 - (5148155107303929*sin(q1L))/9007199254740992))/36893488147419103232)))/2000 - (584133382113593486367040631332731*cos(q6L)*((9007199067919185*((9007199067919185*cos(q4L))/9007199254740992 - (234819211581865*sin(q4L))/1152921504606846976)*((148677514737591106934298605035692608392163854125*cos(q2L))/182687704666362864775460604089535377456991567872 - (127834588709863499538908289888301307693646315855*cos(q1L))/5986310706507378352962293074805895248510699696029696 + (348437586779514700475067630180842053206482623665*sin(q1L))/2993155353253689176481146537402947624255349848014848 + (67682029681889335677290557259385*cos(q2L)*((1888752292310023*cos(q1L))/18014398509481984 - (5148155107303929*sin(q1L))/9007199254740992))/332306998946228968225951765070086144 + (9007199067919185*sin(q2L)*((5148155107303929*cos(q1L))/9007199254740992 + (1888752292310023*sin(q1L))/18014398509481984))/9007199254740992 + 103474418939599489499345508650025439853395886685/3064991081731777716716694054300618367237478244367204352))/9007199254740992 - (9007199067919185*((7514214926474921*cos(q4L))/36893488147419103232 + (4503599440548691*sin(q4L))/4503599627370496)*((9007199067919185*sin(q3L)*((46370457884011341126541404977865*sin(q1L))/81129638414606681695789005144064 - (17012367886825063216155529491255*cos(q1L))/162259276829213363391578010288128 + 13770489658876653055167369550485/83076749736557242056487941267521536))/9007199254740992 - (7514214926474921*sin(q3L)*((16506520352940097956833727997725*cos(q2L))/20282409603651670423947251286016 + (7514214926474921*cos(q2L)*((1888752292310023*cos(q1L))/18014398509481984 - (5148155107303929*sin(q1L))/9007199254740992))/36893488147419103232 + sin(q2L)*((5148155107303929*cos(q1L))/9007199254740992 + (1888752292310023*sin(q1L))/18014398509481984)))/36893488147419103232 + cos(q3L)*((16506520352940097956833727997725*sin(q2L))/20282409603651670423947251286016 - cos(q2L)*((5148155107303929*cos(q1L))/9007199254740992 + (1888752292310023*sin(q1L))/18014398509481984) + (7514214926474921*sin(q2L)*((1888752292310023*cos(q1L))/18014398509481984 - (5148155107303929*sin(q1L))/9007199254740992))/36893488147419103232)))/9007199254740992 + (67682029681889335677290557259385*sin(q4L)*((7514214926474921*cos(q3L)*((16506520352940097956833727997725*cos(q2L))/20282409603651670423947251286016 + (7514214926474921*cos(q2L)*((1888752292310023*cos(q1L))/18014398509481984 - (5148155107303929*sin(q1L))/9007199254740992))/36893488147419103232 + sin(q2L)*((5148155107303929*cos(q1L))/9007199254740992 + (1888752292310023*sin(q1L))/18014398509481984)))/36893488147419103232 - (9007199067919185*cos(q3L)*((46370457884011341126541404977865*sin(q1L))/81129638414606681695789005144064 - (17012367886825063216155529491255*cos(q1L))/162259276829213363391578010288128 + 13770489658876653055167369550485/83076749736557242056487941267521536))/9007199254740992 + sin(q3L)*((16506520352940097956833727997725*sin(q2L))/20282409603651670423947251286016 - cos(q2L)*((5148155107303929*cos(q1L))/9007199254740992 + (1888752292310023*sin(q1L))/18014398509481984) + (7514214926474921*sin(q2L)*((1888752292310023*cos(q1L))/18014398509481984 - (5148155107303929*sin(q1L))/9007199254740992))/36893488147419103232)))/332306998946228968225951765070086144))/16225927682921336339157801028812800 - (48638874966763599*sin(q6L)*((9007199067919185*((9007199067919185*cos(q4L))/9007199254740992 - (234819211581865*sin(q4L))/1152921504606846976)*((148677514737591106934298605035692608392163854125*cos(q2L))/182687704666362864775460604089535377456991567872 - (127834588709863499538908289888301307693646315855*cos(q1L))/5986310706507378352962293074805895248510699696029696 + (348437586779514700475067630180842053206482623665*sin(q1L))/2993155353253689176481146537402947624255349848014848 + (67682029681889335677290557259385*cos(q2L)*((1888752292310023*cos(q1L))/18014398509481984 - (5148155107303929*sin(q1L))/9007199254740992))/332306998946228968225951765070086144 + (9007199067919185*sin(q2L)*((5148155107303929*cos(q1L))/9007199254740992 + (1888752292310023*sin(q1L))/18014398509481984))/9007199254740992 + 103474418939599489499345508650025439853395886685/3064991081731777716716694054300618367237478244367204352))/9007199254740992 - (9007199067919185*((7514214926474921*cos(q4L))/36893488147419103232 + (4503599440548691*sin(q4L))/4503599627370496)*((9007199067919185*sin(q3L)*((46370457884011341126541404977865*sin(q1L))/81129638414606681695789005144064 - (17012367886825063216155529491255*cos(q1L))/162259276829213363391578010288128 + 13770489658876653055167369550485/83076749736557242056487941267521536))/9007199254740992 - (7514214926474921*sin(q3L)*((16506520352940097956833727997725*cos(q2L))/20282409603651670423947251286016 + (7514214926474921*cos(q2L)*((1888752292310023*cos(q1L))/18014398509481984 - (5148155107303929*sin(q1L))/9007199254740992))/36893488147419103232 + sin(q2L)*((5148155107303929*cos(q1L))/9007199254740992 + (1888752292310023*sin(q1L))/18014398509481984)))/36893488147419103232 + cos(q3L)*((16506520352940097956833727997725*sin(q2L))/20282409603651670423947251286016 - cos(q2L)*((5148155107303929*cos(q1L))/9007199254740992 + (1888752292310023*sin(q1L))/18014398509481984) + (7514214926474921*sin(q2L)*((1888752292310023*cos(q1L))/18014398509481984 - (5148155107303929*sin(q1L))/9007199254740992))/36893488147419103232)))/9007199254740992 + (67682029681889335677290557259385*sin(q4L)*((7514214926474921*cos(q3L)*((16506520352940097956833727997725*cos(q2L))/20282409603651670423947251286016 + (7514214926474921*cos(q2L)*((1888752292310023*cos(q1L))/18014398509481984 - (5148155107303929*sin(q1L))/9007199254740992))/36893488147419103232 + sin(q2L)*((5148155107303929*cos(q1L))/9007199254740992 + (1888752292310023*sin(q1L))/18014398509481984)))/36893488147419103232 - (9007199067919185*cos(q3L)*((46370457884011341126541404977865*sin(q1L))/81129638414606681695789005144064 - (17012367886825063216155529491255*cos(q1L))/162259276829213363391578010288128 + 13770489658876653055167369550485/83076749736557242056487941267521536))/9007199254740992 + sin(q3L)*((16506520352940097956833727997725*sin(q2L))/20282409603651670423947251286016 - cos(q2L)*((5148155107303929*cos(q1L))/9007199254740992 + (1888752292310023*sin(q1L))/18014398509481984) + (7514214926474921*sin(q2L)*((1888752292310023*cos(q1L))/18014398509481984 - (5148155107303929*sin(q1L))/9007199254740992))/36893488147419103232)))/332306998946228968225951765070086144))/1801439850948198400 - (27*cos(q6L)*(cos(q5L)*(((4503599440548691*cos(q4L))/4503599627370496 - (7514214926474921*sin(q4L))/36893488147419103232)*((9007199067919185*sin(q3L)*((46370457884011341126541404977865*sin(q1L))/81129638414606681695789005144064 - (17012367886825063216155529491255*cos(q1L))/162259276829213363391578010288128 + 13770489658876653055167369550485/83076749736557242056487941267521536))/9007199254740992 - (7514214926474921*sin(q3L)*((16506520352940097956833727997725*cos(q2L))/20282409603651670423947251286016 + (7514214926474921*cos(q2L)*((1888752292310023*cos(q1L))/18014398509481984 - (5148155107303929*sin(q1L))/9007199254740992))/36893488147419103232 + sin(q2L)*((5148155107303929*cos(q1L))/9007199254740992 + (1888752292310023*sin(q1L))/18014398509481984)))/36893488147419103232 + cos(q3L)*((16506520352940097956833727997725*sin(q2L))/20282409603651670423947251286016 - cos(q2L)*((5148155107303929*cos(q1L))/9007199254740992 + (1888752292310023*sin(q1L))/18014398509481984) + (7514214926474921*sin(q2L)*((1888752292310023*cos(q1L))/18014398509481984 - (5148155107303929*sin(q1L))/9007199254740992))/36893488147419103232)) + ((234819211581865*cos(q4L))/1152921504606846976 + (9007199067919185*sin(q4L))/9007199254740992)*((148677514737591106934298605035692608392163854125*cos(q2L))/182687704666362864775460604089535377456991567872 - (127834588709863499538908289888301307693646315855*cos(q1L))/5986310706507378352962293074805895248510699696029696 + (348437586779514700475067630180842053206482623665*sin(q1L))/2993155353253689176481146537402947624255349848014848 + (67682029681889335677290557259385*cos(q2L)*((1888752292310023*cos(q1L))/18014398509481984 - (5148155107303929*sin(q1L))/9007199254740992))/332306998946228968225951765070086144 + (9007199067919185*sin(q2L)*((5148155107303929*cos(q1L))/9007199254740992 + (1888752292310023*sin(q1L))/18014398509481984))/9007199254740992 + 103474418939599489499345508650025439853395886685/3064991081731777716716694054300618367237478244367204352) - (7514214926474921*cos(q4L)*((7514214926474921*cos(q3L)*((16506520352940097956833727997725*cos(q2L))/20282409603651670423947251286016 + (7514214926474921*cos(q2L)*((1888752292310023*cos(q1L))/18014398509481984 - (5148155107303929*sin(q1L))/9007199254740992))/36893488147419103232 + sin(q2L)*((5148155107303929*cos(q1L))/9007199254740992 + (1888752292310023*sin(q1L))/18014398509481984)))/36893488147419103232 - (9007199067919185*cos(q3L)*((46370457884011341126541404977865*sin(q1L))/81129638414606681695789005144064 - (17012367886825063216155529491255*cos(q1L))/162259276829213363391578010288128 + 13770489658876653055167369550485/83076749736557242056487941267521536))/9007199254740992 + sin(q3L)*((16506520352940097956833727997725*sin(q2L))/20282409603651670423947251286016 - cos(q2L)*((5148155107303929*cos(q1L))/9007199254740992 + (1888752292310023*sin(q1L))/18014398509481984) + (7514214926474921*sin(q2L)*((1888752292310023*cos(q1L))/18014398509481984 - (5148155107303929*sin(q1L))/9007199254740992))/36893488147419103232)))/36893488147419103232) - (7514214926474921*sin(q5L)*(((9007199067919185*cos(q4L))/9007199254740992 - (234819211581865*sin(q4L))/1152921504606846976)*((148677514737591106934298605035692608392163854125*cos(q2L))/182687704666362864775460604089535377456991567872 - (127834588709863499538908289888301307693646315855*cos(q1L))/5986310706507378352962293074805895248510699696029696 + (348437586779514700475067630180842053206482623665*sin(q1L))/2993155353253689176481146537402947624255349848014848 + (67682029681889335677290557259385*cos(q2L)*((1888752292310023*cos(q1L))/18014398509481984 - (5148155107303929*sin(q1L))/9007199254740992))/332306998946228968225951765070086144 + (9007199067919185*sin(q2L)*((5148155107303929*cos(q1L))/9007199254740992 + (1888752292310023*sin(q1L))/18014398509481984))/9007199254740992 + 103474418939599489499345508650025439853395886685/3064991081731777716716694054300618367237478244367204352) - ((7514214926474921*cos(q4L))/36893488147419103232 + (4503599440548691*sin(q4L))/4503599627370496)*((9007199067919185*sin(q3L)*((46370457884011341126541404977865*sin(q1L))/81129638414606681695789005144064 - (17012367886825063216155529491255*cos(q1L))/162259276829213363391578010288128 + 13770489658876653055167369550485/83076749736557242056487941267521536))/9007199254740992 - (7514214926474921*sin(q3L)*((16506520352940097956833727997725*cos(q2L))/20282409603651670423947251286016 + (7514214926474921*cos(q2L)*((1888752292310023*cos(q1L))/18014398509481984 - (5148155107303929*sin(q1L))/9007199254740992))/36893488147419103232 + sin(q2L)*((5148155107303929*cos(q1L))/9007199254740992 + (1888752292310023*sin(q1L))/18014398509481984)))/36893488147419103232 + cos(q3L)*((16506520352940097956833727997725*sin(q2L))/20282409603651670423947251286016 - cos(q2L)*((5148155107303929*cos(q1L))/9007199254740992 + (1888752292310023*sin(q1L))/18014398509481984) + (7514214926474921*sin(q2L)*((1888752292310023*cos(q1L))/18014398509481984 - (5148155107303929*sin(q1L))/9007199254740992))/36893488147419103232)) + (7514214926474921*sin(q4L)*((7514214926474921*cos(q3L)*((16506520352940097956833727997725*cos(q2L))/20282409603651670423947251286016 + (7514214926474921*cos(q2L)*((1888752292310023*cos(q1L))/18014398509481984 - (5148155107303929*sin(q1L))/9007199254740992))/36893488147419103232 + sin(q2L)*((5148155107303929*cos(q1L))/9007199254740992 + (1888752292310023*sin(q1L))/18014398509481984)))/36893488147419103232 - (9007199067919185*cos(q3L)*((46370457884011341126541404977865*sin(q1L))/81129638414606681695789005144064 - (17012367886825063216155529491255*cos(q1L))/162259276829213363391578010288128 + 13770489658876653055167369550485/83076749736557242056487941267521536))/9007199254740992 + sin(q3L)*((16506520352940097956833727997725*sin(q2L))/20282409603651670423947251286016 - cos(q2L)*((5148155107303929*cos(q1L))/9007199254740992 + (1888752292310023*sin(q1L))/18014398509481984) + (7514214926474921*sin(q2L)*((1888752292310023*cos(q1L))/18014398509481984 - (5148155107303929*sin(q1L))/9007199254740992))/36893488147419103232)))/36893488147419103232))/36893488147419103232))/1000 - (2436553109258773196144549622003023*cos(q6L)*(sin(q5L)*(((4503599440548691*cos(q4L))/4503599627370496 - (7514214926474921*sin(q4L))/36893488147419103232)*((9007199067919185*sin(q3L)*((46370457884011341126541404977865*sin(q1L))/81129638414606681695789005144064 - (17012367886825063216155529491255*cos(q1L))/162259276829213363391578010288128 + 13770489658876653055167369550485/83076749736557242056487941267521536))/9007199254740992 - (7514214926474921*sin(q3L)*((16506520352940097956833727997725*cos(q2L))/20282409603651670423947251286016 + (7514214926474921*cos(q2L)*((1888752292310023*cos(q1L))/18014398509481984 - (5148155107303929*sin(q1L))/9007199254740992))/36893488147419103232 + sin(q2L)*((5148155107303929*cos(q1L))/9007199254740992 + (1888752292310023*sin(q1L))/18014398509481984)))/36893488147419103232 + cos(q3L)*((16506520352940097956833727997725*sin(q2L))/20282409603651670423947251286016 - cos(q2L)*((5148155107303929*cos(q1L))/9007199254740992 + (1888752292310023*sin(q1L))/18014398509481984) + (7514214926474921*sin(q2L)*((1888752292310023*cos(q1L))/18014398509481984 - (5148155107303929*sin(q1L))/9007199254740992))/36893488147419103232)) + ((234819211581865*cos(q4L))/1152921504606846976 + (9007199067919185*sin(q4L))/9007199254740992)*((148677514737591106934298605035692608392163854125*cos(q2L))/182687704666362864775460604089535377456991567872 - (127834588709863499538908289888301307693646315855*cos(q1L))/5986310706507378352962293074805895248510699696029696 + (348437586779514700475067630180842053206482623665*sin(q1L))/2993155353253689176481146537402947624255349848014848 + (67682029681889335677290557259385*cos(q2L)*((1888752292310023*cos(q1L))/18014398509481984 - (5148155107303929*sin(q1L))/9007199254740992))/332306998946228968225951765070086144 + (9007199067919185*sin(q2L)*((5148155107303929*cos(q1L))/9007199254740992 + (1888752292310023*sin(q1L))/18014398509481984))/9007199254740992 + 103474418939599489499345508650025439853395886685/3064991081731777716716694054300618367237478244367204352) - (7514214926474921*cos(q4L)*((7514214926474921*cos(q3L)*((16506520352940097956833727997725*cos(q2L))/20282409603651670423947251286016 + (7514214926474921*cos(q2L)*((1888752292310023*cos(q1L))/18014398509481984 - (5148155107303929*sin(q1L))/9007199254740992))/36893488147419103232 + sin(q2L)*((5148155107303929*cos(q1L))/9007199254740992 + (1888752292310023*sin(q1L))/18014398509481984)))/36893488147419103232 - (9007199067919185*cos(q3L)*((46370457884011341126541404977865*sin(q1L))/81129638414606681695789005144064 - (17012367886825063216155529491255*cos(q1L))/162259276829213363391578010288128 + 13770489658876653055167369550485/83076749736557242056487941267521536))/9007199254740992 + sin(q3L)*((16506520352940097956833727997725*sin(q2L))/20282409603651670423947251286016 - cos(q2L)*((5148155107303929*cos(q1L))/9007199254740992 + (1888752292310023*sin(q1L))/18014398509481984) + (7514214926474921*sin(q2L)*((1888752292310023*cos(q1L))/18014398509481984 - (5148155107303929*sin(q1L))/9007199254740992))/36893488147419103232)))/36893488147419103232) + (7514214926474921*cos(q5L)*(((9007199067919185*cos(q4L))/9007199254740992 - (234819211581865*sin(q4L))/1152921504606846976)*((148677514737591106934298605035692608392163854125*cos(q2L))/182687704666362864775460604089535377456991567872 - (127834588709863499538908289888301307693646315855*cos(q1L))/5986310706507378352962293074805895248510699696029696 + (348437586779514700475067630180842053206482623665*sin(q1L))/2993155353253689176481146537402947624255349848014848 + (67682029681889335677290557259385*cos(q2L)*((1888752292310023*cos(q1L))/18014398509481984 - (5148155107303929*sin(q1L))/9007199254740992))/332306998946228968225951765070086144 + (9007199067919185*sin(q2L)*((5148155107303929*cos(q1L))/9007199254740992 + (1888752292310023*sin(q1L))/18014398509481984))/9007199254740992 + 103474418939599489499345508650025439853395886685/3064991081731777716716694054300618367237478244367204352) - ((7514214926474921*cos(q4L))/36893488147419103232 + (4503599440548691*sin(q4L))/4503599627370496)*((9007199067919185*sin(q3L)*((46370457884011341126541404977865*sin(q1L))/81129638414606681695789005144064 - (17012367886825063216155529491255*cos(q1L))/162259276829213363391578010288128 + 13770489658876653055167369550485/83076749736557242056487941267521536))/9007199254740992 - (7514214926474921*sin(q3L)*((16506520352940097956833727997725*cos(q2L))/20282409603651670423947251286016 + (7514214926474921*cos(q2L)*((1888752292310023*cos(q1L))/18014398509481984 - (5148155107303929*sin(q1L))/9007199254740992))/36893488147419103232 + sin(q2L)*((5148155107303929*cos(q1L))/9007199254740992 + (1888752292310023*sin(q1L))/18014398509481984)))/36893488147419103232 + cos(q3L)*((16506520352940097956833727997725*sin(q2L))/20282409603651670423947251286016 - cos(q2L)*((5148155107303929*cos(q1L))/9007199254740992 + (1888752292310023*sin(q1L))/18014398509481984) + (7514214926474921*sin(q2L)*((1888752292310023*cos(q1L))/18014398509481984 - (5148155107303929*sin(q1L))/9007199254740992))/36893488147419103232)) + (7514214926474921*sin(q4L)*((7514214926474921*cos(q3L)*((16506520352940097956833727997725*cos(q2L))/20282409603651670423947251286016 + (7514214926474921*cos(q2L)*((1888752292310023*cos(q1L))/18014398509481984 - (5148155107303929*sin(q1L))/9007199254740992))/36893488147419103232 + sin(q2L)*((5148155107303929*cos(q1L))/9007199254740992 + (1888752292310023*sin(q1L))/18014398509481984)))/36893488147419103232 - (9007199067919185*cos(q3L)*((46370457884011341126541404977865*sin(q1L))/81129638414606681695789005144064 - (17012367886825063216155529491255*cos(q1L))/162259276829213363391578010288128 + 13770489658876653055167369550485/83076749736557242056487941267521536))/9007199254740992 + sin(q3L)*((16506520352940097956833727997725*sin(q2L))/20282409603651670423947251286016 - cos(q2L)*((5148155107303929*cos(q1L))/9007199254740992 + (1888752292310023*sin(q1L))/18014398509481984) + (7514214926474921*sin(q2L)*((1888752292310023*cos(q1L))/18014398509481984 - (5148155107303929*sin(q1L))/9007199254740992))/36893488147419103232)))/36893488147419103232))/36893488147419103232))/332306998946228968225951765070086144000 + (324259171862923063*sin(q6L)*(cos(q5L)*(((4503599440548691*cos(q4L))/4503599627370496 - (7514214926474921*sin(q4L))/36893488147419103232)*((9007199067919185*sin(q3L)*((46370457884011341126541404977865*sin(q1L))/81129638414606681695789005144064 - (17012367886825063216155529491255*cos(q1L))/162259276829213363391578010288128 + 13770489658876653055167369550485/83076749736557242056487941267521536))/9007199254740992 - (7514214926474921*sin(q3L)*((16506520352940097956833727997725*cos(q2L))/20282409603651670423947251286016 + (7514214926474921*cos(q2L)*((1888752292310023*cos(q1L))/18014398509481984 - (5148155107303929*sin(q1L))/9007199254740992))/36893488147419103232 + sin(q2L)*((5148155107303929*cos(q1L))/9007199254740992 + (1888752292310023*sin(q1L))/18014398509481984)))/36893488147419103232 + cos(q3L)*((16506520352940097956833727997725*sin(q2L))/20282409603651670423947251286016 - cos(q2L)*((5148155107303929*cos(q1L))/9007199254740992 + (1888752292310023*sin(q1L))/18014398509481984) + (7514214926474921*sin(q2L)*((1888752292310023*cos(q1L))/18014398509481984 - (5148155107303929*sin(q1L))/9007199254740992))/36893488147419103232)) + ((234819211581865*cos(q4L))/1152921504606846976 + (9007199067919185*sin(q4L))/9007199254740992)*((148677514737591106934298605035692608392163854125*cos(q2L))/182687704666362864775460604089535377456991567872 - (127834588709863499538908289888301307693646315855*cos(q1L))/5986310706507378352962293074805895248510699696029696 + (348437586779514700475067630180842053206482623665*sin(q1L))/2993155353253689176481146537402947624255349848014848 + (67682029681889335677290557259385*cos(q2L)*((1888752292310023*cos(q1L))/18014398509481984 - (5148155107303929*sin(q1L))/9007199254740992))/332306998946228968225951765070086144 + (9007199067919185*sin(q2L)*((5148155107303929*cos(q1L))/9007199254740992 + (1888752292310023*sin(q1L))/18014398509481984))/9007199254740992 + 103474418939599489499345508650025439853395886685/3064991081731777716716694054300618367237478244367204352) - (7514214926474921*cos(q4L)*((7514214926474921*cos(q3L)*((16506520352940097956833727997725*cos(q2L))/20282409603651670423947251286016 + (7514214926474921*cos(q2L)*((1888752292310023*cos(q1L))/18014398509481984 - (5148155107303929*sin(q1L))/9007199254740992))/36893488147419103232 + sin(q2L)*((5148155107303929*cos(q1L))/9007199254740992 + (1888752292310023*sin(q1L))/18014398509481984)))/36893488147419103232 - (9007199067919185*cos(q3L)*((46370457884011341126541404977865*sin(q1L))/81129638414606681695789005144064 - (17012367886825063216155529491255*cos(q1L))/162259276829213363391578010288128 + 13770489658876653055167369550485/83076749736557242056487941267521536))/9007199254740992 + sin(q3L)*((16506520352940097956833727997725*sin(q2L))/20282409603651670423947251286016 - cos(q2L)*((5148155107303929*cos(q1L))/9007199254740992 + (1888752292310023*sin(q1L))/18014398509481984) + (7514214926474921*sin(q2L)*((1888752292310023*cos(q1L))/18014398509481984 - (5148155107303929*sin(q1L))/9007199254740992))/36893488147419103232)))/36893488147419103232) - (7514214926474921*sin(q5L)*(((9007199067919185*cos(q4L))/9007199254740992 - (234819211581865*sin(q4L))/1152921504606846976)*((148677514737591106934298605035692608392163854125*cos(q2L))/182687704666362864775460604089535377456991567872 - (127834588709863499538908289888301307693646315855*cos(q1L))/5986310706507378352962293074805895248510699696029696 + (348437586779514700475067630180842053206482623665*sin(q1L))/2993155353253689176481146537402947624255349848014848 + (67682029681889335677290557259385*cos(q2L)*((1888752292310023*cos(q1L))/18014398509481984 - (5148155107303929*sin(q1L))/9007199254740992))/332306998946228968225951765070086144 + (9007199067919185*sin(q2L)*((5148155107303929*cos(q1L))/9007199254740992 + (1888752292310023*sin(q1L))/18014398509481984))/9007199254740992 + 103474418939599489499345508650025439853395886685/3064991081731777716716694054300618367237478244367204352) - ((7514214926474921*cos(q4L))/36893488147419103232 + (4503599440548691*sin(q4L))/4503599627370496)*((9007199067919185*sin(q3L)*((46370457884011341126541404977865*sin(q1L))/81129638414606681695789005144064 - (17012367886825063216155529491255*cos(q1L))/162259276829213363391578010288128 + 13770489658876653055167369550485/83076749736557242056487941267521536))/9007199254740992 - (7514214926474921*sin(q3L)*((16506520352940097956833727997725*cos(q2L))/20282409603651670423947251286016 + (7514214926474921*cos(q2L)*((1888752292310023*cos(q1L))/18014398509481984 - (5148155107303929*sin(q1L))/9007199254740992))/36893488147419103232 + sin(q2L)*((5148155107303929*cos(q1L))/9007199254740992 + (1888752292310023*sin(q1L))/18014398509481984)))/36893488147419103232 + cos(q3L)*((16506520352940097956833727997725*sin(q2L))/20282409603651670423947251286016 - cos(q2L)*((5148155107303929*cos(q1L))/9007199254740992 + (1888752292310023*sin(q1L))/18014398509481984) + (7514214926474921*sin(q2L)*((1888752292310023*cos(q1L))/18014398509481984 - (5148155107303929*sin(q1L))/9007199254740992))/36893488147419103232)) + (7514214926474921*sin(q4L)*((7514214926474921*cos(q3L)*((16506520352940097956833727997725*cos(q2L))/20282409603651670423947251286016 + (7514214926474921*cos(q2L)*((1888752292310023*cos(q1L))/18014398509481984 - (5148155107303929*sin(q1L))/9007199254740992))/36893488147419103232 + sin(q2L)*((5148155107303929*cos(q1L))/9007199254740992 + (1888752292310023*sin(q1L))/18014398509481984)))/36893488147419103232 - (9007199067919185*cos(q3L)*((46370457884011341126541404977865*sin(q1L))/81129638414606681695789005144064 - (17012367886825063216155529491255*cos(q1L))/162259276829213363391578010288128 + 13770489658876653055167369550485/83076749736557242056487941267521536))/9007199254740992 + sin(q3L)*((16506520352940097956833727997725*sin(q2L))/20282409603651670423947251286016 - cos(q2L)*((5148155107303929*cos(q1L))/9007199254740992 + (1888752292310023*sin(q1L))/18014398509481984) + (7514214926474921*sin(q2L)*((1888752292310023*cos(q1L))/18014398509481984 - (5148155107303929*sin(q1L))/9007199254740992))/36893488147419103232)))/36893488147419103232))/36893488147419103232))/9007199254740992000 - (202883803014822867*sin(q6L)*(sin(q5L)*(((4503599440548691*cos(q4L))/4503599627370496 - (7514214926474921*sin(q4L))/36893488147419103232)*((9007199067919185*sin(q3L)*((46370457884011341126541404977865*sin(q1L))/81129638414606681695789005144064 - (17012367886825063216155529491255*cos(q1L))/162259276829213363391578010288128 + 13770489658876653055167369550485/83076749736557242056487941267521536))/9007199254740992 - (7514214926474921*sin(q3L)*((16506520352940097956833727997725*cos(q2L))/20282409603651670423947251286016 + (7514214926474921*cos(q2L)*((1888752292310023*cos(q1L))/18014398509481984 - (5148155107303929*sin(q1L))/9007199254740992))/36893488147419103232 + sin(q2L)*((5148155107303929*cos(q1L))/9007199254740992 + (1888752292310023*sin(q1L))/18014398509481984)))/36893488147419103232 + cos(q3L)*((16506520352940097956833727997725*sin(q2L))/20282409603651670423947251286016 - cos(q2L)*((5148155107303929*cos(q1L))/9007199254740992 + (1888752292310023*sin(q1L))/18014398509481984) + (7514214926474921*sin(q2L)*((1888752292310023*cos(q1L))/18014398509481984 - (5148155107303929*sin(q1L))/9007199254740992))/36893488147419103232)) + ((234819211581865*cos(q4L))/1152921504606846976 + (9007199067919185*sin(q4L))/9007199254740992)*((148677514737591106934298605035692608392163854125*cos(q2L))/182687704666362864775460604089535377456991567872 - (127834588709863499538908289888301307693646315855*cos(q1L))/5986310706507378352962293074805895248510699696029696 + (348437586779514700475067630180842053206482623665*sin(q1L))/2993155353253689176481146537402947624255349848014848 + (67682029681889335677290557259385*cos(q2L)*((1888752292310023*cos(q1L))/18014398509481984 - (5148155107303929*sin(q1L))/9007199254740992))/332306998946228968225951765070086144 + (9007199067919185*sin(q2L)*((5148155107303929*cos(q1L))/9007199254740992 + (1888752292310023*sin(q1L))/18014398509481984))/9007199254740992 + 103474418939599489499345508650025439853395886685/3064991081731777716716694054300618367237478244367204352) - (7514214926474921*cos(q4L)*((7514214926474921*cos(q3L)*((16506520352940097956833727997725*cos(q2L))/20282409603651670423947251286016 + (7514214926474921*cos(q2L)*((1888752292310023*cos(q1L))/18014398509481984 - (5148155107303929*sin(q1L))/9007199254740992))/36893488147419103232 + sin(q2L)*((5148155107303929*cos(q1L))/9007199254740992 + (1888752292310023*sin(q1L))/18014398509481984)))/36893488147419103232 - (9007199067919185*cos(q3L)*((46370457884011341126541404977865*sin(q1L))/81129638414606681695789005144064 - (17012367886825063216155529491255*cos(q1L))/162259276829213363391578010288128 + 13770489658876653055167369550485/83076749736557242056487941267521536))/9007199254740992 + sin(q3L)*((16506520352940097956833727997725*sin(q2L))/20282409603651670423947251286016 - cos(q2L)*((5148155107303929*cos(q1L))/9007199254740992 + (1888752292310023*sin(q1L))/18014398509481984) + (7514214926474921*sin(q2L)*((1888752292310023*cos(q1L))/18014398509481984 - (5148155107303929*sin(q1L))/9007199254740992))/36893488147419103232)))/36893488147419103232) + (7514214926474921*cos(q5L)*(((9007199067919185*cos(q4L))/9007199254740992 - (234819211581865*sin(q4L))/1152921504606846976)*((148677514737591106934298605035692608392163854125*cos(q2L))/182687704666362864775460604089535377456991567872 - (127834588709863499538908289888301307693646315855*cos(q1L))/5986310706507378352962293074805895248510699696029696 + (348437586779514700475067630180842053206482623665*sin(q1L))/2993155353253689176481146537402947624255349848014848 + (67682029681889335677290557259385*cos(q2L)*((1888752292310023*cos(q1L))/18014398509481984 - (5148155107303929*sin(q1L))/9007199254740992))/332306998946228968225951765070086144 + (9007199067919185*sin(q2L)*((5148155107303929*cos(q1L))/9007199254740992 + (1888752292310023*sin(q1L))/18014398509481984))/9007199254740992 + 103474418939599489499345508650025439853395886685/3064991081731777716716694054300618367237478244367204352) - ((7514214926474921*cos(q4L))/36893488147419103232 + (4503599440548691*sin(q4L))/4503599627370496)*((9007199067919185*sin(q3L)*((46370457884011341126541404977865*sin(q1L))/81129638414606681695789005144064 - (17012367886825063216155529491255*cos(q1L))/162259276829213363391578010288128 + 13770489658876653055167369550485/83076749736557242056487941267521536))/9007199254740992 - (7514214926474921*sin(q3L)*((16506520352940097956833727997725*cos(q2L))/20282409603651670423947251286016 + (7514214926474921*cos(q2L)*((1888752292310023*cos(q1L))/18014398509481984 - (5148155107303929*sin(q1L))/9007199254740992))/36893488147419103232 + sin(q2L)*((5148155107303929*cos(q1L))/9007199254740992 + (1888752292310023*sin(q1L))/18014398509481984)))/36893488147419103232 + cos(q3L)*((16506520352940097956833727997725*sin(q2L))/20282409603651670423947251286016 - cos(q2L)*((5148155107303929*cos(q1L))/9007199254740992 + (1888752292310023*sin(q1L))/18014398509481984) + (7514214926474921*sin(q2L)*((1888752292310023*cos(q1L))/18014398509481984 - (5148155107303929*sin(q1L))/9007199254740992))/36893488147419103232)) + (7514214926474921*sin(q4L)*((7514214926474921*cos(q3L)*((16506520352940097956833727997725*cos(q2L))/20282409603651670423947251286016 + (7514214926474921*cos(q2L)*((1888752292310023*cos(q1L))/18014398509481984 - (5148155107303929*sin(q1L))/9007199254740992))/36893488147419103232 + sin(q2L)*((5148155107303929*cos(q1L))/9007199254740992 + (1888752292310023*sin(q1L))/18014398509481984)))/36893488147419103232 - (9007199067919185*cos(q3L)*((46370457884011341126541404977865*sin(q1L))/81129638414606681695789005144064 - (17012367886825063216155529491255*cos(q1L))/162259276829213363391578010288128 + 13770489658876653055167369550485/83076749736557242056487941267521536))/9007199254740992 + sin(q3L)*((16506520352940097956833727997725*sin(q2L))/20282409603651670423947251286016 - cos(q2L)*((5148155107303929*cos(q1L))/9007199254740992 + (1888752292310023*sin(q1L))/18014398509481984) + (7514214926474921*sin(q2L)*((1888752292310023*cos(q1L))/18014398509481984 - (5148155107303929*sin(q1L))/9007199254740992))/36893488147419103232)))/36893488147419103232))/36893488147419103232))/36893488147419103232000 - (81222263116692158804177042061221826384594597321566869716687*((9007199067919185*cos(q4L))/9007199254740992 - (234819211581865*sin(q4L))/1152921504606846976)*((148677514737591106934298605035692608392163854125*cos(q2L))/182687704666362864775460604089535377456991567872 - (127834588709863499538908289888301307693646315855*cos(q1L))/5986310706507378352962293074805895248510699696029696 + (348437586779514700475067630180842053206482623665*sin(q1L))/2993155353253689176481146537402947624255349848014848 + (67682029681889335677290557259385*cos(q2L)*((1888752292310023*cos(q1L))/18014398509481984 - (5148155107303929*sin(q1L))/9007199254740992))/332306998946228968225951765070086144 + (9007199067919185*sin(q2L)*((5148155107303929*cos(q1L))/9007199254740992 + (1888752292310023*sin(q1L))/18014398509481984))/9007199254740992 + 103474418939599489499345508650025439853395886685/3064991081731777716716694054300618367237478244367204352))/306499108173177771671669405430061836723747824436720435200000 - (81*((234819211581865*cos(q4L))/1152921504606846976 + (9007199067919185*sin(q4L))/9007199254740992)*((148677514737591106934298605035692608392163854125*cos(q2L))/182687704666362864775460604089535377456991567872 - (127834588709863499538908289888301307693646315855*cos(q1L))/5986310706507378352962293074805895248510699696029696 + (348437586779514700475067630180842053206482623665*sin(q1L))/2993155353253689176481146537402947624255349848014848 + (67682029681889335677290557259385*cos(q2L)*((1888752292310023*cos(q1L))/18014398509481984 - (5148155107303929*sin(q1L))/9007199254740992))/332306998946228968225951765070086144 + (9007199067919185*sin(q2L)*((5148155107303929*cos(q1L))/9007199254740992 + (1888752292310023*sin(q1L))/18014398509481984))/9007199254740992 + 103474418939599489499345508650025439853395886685/3064991081731777716716694054300618367237478244367204352))/2000 + (27*cos(q5L)*(((4503599440548691*cos(q4L))/4503599627370496 - (7514214926474921*sin(q4L))/36893488147419103232)*((9007199067919185*sin(q3L)*((46370457884011341126541404977865*sin(q1L))/81129638414606681695789005144064 - (17012367886825063216155529491255*cos(q1L))/162259276829213363391578010288128 + 13770489658876653055167369550485/83076749736557242056487941267521536))/9007199254740992 - (7514214926474921*sin(q3L)*((16506520352940097956833727997725*cos(q2L))/20282409603651670423947251286016 + (7514214926474921*cos(q2L)*((1888752292310023*cos(q1L))/18014398509481984 - (5148155107303929*sin(q1L))/9007199254740992))/36893488147419103232 + sin(q2L)*((5148155107303929*cos(q1L))/9007199254740992 + (1888752292310023*sin(q1L))/18014398509481984)))/36893488147419103232 + cos(q3L)*((16506520352940097956833727997725*sin(q2L))/20282409603651670423947251286016 - cos(q2L)*((5148155107303929*cos(q1L))/9007199254740992 + (1888752292310023*sin(q1L))/18014398509481984) + (7514214926474921*sin(q2L)*((1888752292310023*cos(q1L))/18014398509481984 - (5148155107303929*sin(q1L))/9007199254740992))/36893488147419103232)) + ((234819211581865*cos(q4L))/1152921504606846976 + (9007199067919185*sin(q4L))/9007199254740992)*((148677514737591106934298605035692608392163854125*cos(q2L))/182687704666362864775460604089535377456991567872 - (127834588709863499538908289888301307693646315855*cos(q1L))/5986310706507378352962293074805895248510699696029696 + (348437586779514700475067630180842053206482623665*sin(q1L))/2993155353253689176481146537402947624255349848014848 + (67682029681889335677290557259385*cos(q2L)*((1888752292310023*cos(q1L))/18014398509481984 - (5148155107303929*sin(q1L))/9007199254740992))/332306998946228968225951765070086144 + (9007199067919185*sin(q2L)*((5148155107303929*cos(q1L))/9007199254740992 + (1888752292310023*sin(q1L))/18014398509481984))/9007199254740992 + 103474418939599489499345508650025439853395886685/3064991081731777716716694054300618367237478244367204352) - (7514214926474921*cos(q4L)*((7514214926474921*cos(q3L)*((16506520352940097956833727997725*cos(q2L))/20282409603651670423947251286016 + (7514214926474921*cos(q2L)*((1888752292310023*cos(q1L))/18014398509481984 - (5148155107303929*sin(q1L))/9007199254740992))/36893488147419103232 + sin(q2L)*((5148155107303929*cos(q1L))/9007199254740992 + (1888752292310023*sin(q1L))/18014398509481984)))/36893488147419103232 - (9007199067919185*cos(q3L)*((46370457884011341126541404977865*sin(q1L))/81129638414606681695789005144064 - (17012367886825063216155529491255*cos(q1L))/162259276829213363391578010288128 + 13770489658876653055167369550485/83076749736557242056487941267521536))/9007199254740992 + sin(q3L)*((16506520352940097956833727997725*sin(q2L))/20282409603651670423947251286016 - cos(q2L)*((5148155107303929*cos(q1L))/9007199254740992 + (1888752292310023*sin(q1L))/18014398509481984) + (7514214926474921*sin(q2L)*((1888752292310023*cos(q1L))/18014398509481984 - (5148155107303929*sin(q1L))/9007199254740992))/36893488147419103232)))/36893488147419103232))/1000 + (94754841554645069948206780163139*sin(q5L)*(((4503599440548691*cos(q4L))/4503599627370496 - (7514214926474921*sin(q4L))/36893488147419103232)*((9007199067919185*sin(q3L)*((46370457884011341126541404977865*sin(q1L))/81129638414606681695789005144064 - (17012367886825063216155529491255*cos(q1L))/162259276829213363391578010288128 + 13770489658876653055167369550485/83076749736557242056487941267521536))/9007199254740992 - (7514214926474921*sin(q3L)*((16506520352940097956833727997725*cos(q2L))/20282409603651670423947251286016 + (7514214926474921*cos(q2L)*((1888752292310023*cos(q1L))/18014398509481984 - (5148155107303929*sin(q1L))/9007199254740992))/36893488147419103232 + sin(q2L)*((5148155107303929*cos(q1L))/9007199254740992 + (1888752292310023*sin(q1L))/18014398509481984)))/36893488147419103232 + cos(q3L)*((16506520352940097956833727997725*sin(q2L))/20282409603651670423947251286016 - cos(q2L)*((5148155107303929*cos(q1L))/9007199254740992 + (1888752292310023*sin(q1L))/18014398509481984) + (7514214926474921*sin(q2L)*((1888752292310023*cos(q1L))/18014398509481984 - (5148155107303929*sin(q1L))/9007199254740992))/36893488147419103232)) + ((234819211581865*cos(q4L))/1152921504606846976 + (9007199067919185*sin(q4L))/9007199254740992)*((148677514737591106934298605035692608392163854125*cos(q2L))/182687704666362864775460604089535377456991567872 - (127834588709863499538908289888301307693646315855*cos(q1L))/5986310706507378352962293074805895248510699696029696 + (348437586779514700475067630180842053206482623665*sin(q1L))/2993155353253689176481146537402947624255349848014848 + (67682029681889335677290557259385*cos(q2L)*((1888752292310023*cos(q1L))/18014398509481984 - (5148155107303929*sin(q1L))/9007199254740992))/332306998946228968225951765070086144 + (9007199067919185*sin(q2L)*((5148155107303929*cos(q1L))/9007199254740992 + (1888752292310023*sin(q1L))/18014398509481984))/9007199254740992 + 103474418939599489499345508650025439853395886685/3064991081731777716716694054300618367237478244367204352) - (7514214926474921*cos(q4L)*((7514214926474921*cos(q3L)*((16506520352940097956833727997725*cos(q2L))/20282409603651670423947251286016 + (7514214926474921*cos(q2L)*((1888752292310023*cos(q1L))/18014398509481984 - (5148155107303929*sin(q1L))/9007199254740992))/36893488147419103232 + sin(q2L)*((5148155107303929*cos(q1L))/9007199254740992 + (1888752292310023*sin(q1L))/18014398509481984)))/36893488147419103232 - (9007199067919185*cos(q3L)*((46370457884011341126541404977865*sin(q1L))/81129638414606681695789005144064 - (17012367886825063216155529491255*cos(q1L))/162259276829213363391578010288128 + 13770489658876653055167369550485/83076749736557242056487941267521536))/9007199254740992 + sin(q3L)*((16506520352940097956833727997725*sin(q2L))/20282409603651670423947251286016 - cos(q2L)*((5148155107303929*cos(q1L))/9007199254740992 + (1888752292310023*sin(q1L))/18014398509481984) + (7514214926474921*sin(q2L)*((1888752292310023*cos(q1L))/18014398509481984 - (5148155107303929*sin(q1L))/9007199254740992))/36893488147419103232)))/36893488147419103232))/66461399789245793645190353014017228800 + (712008244765680093343103025701132101054572137019*cos(q5L)*(((9007199067919185*cos(q4L))/9007199254740992 - (234819211581865*sin(q4L))/1152921504606846976)*((148677514737591106934298605035692608392163854125*cos(q2L))/182687704666362864775460604089535377456991567872 - (127834588709863499538908289888301307693646315855*cos(q1L))/5986310706507378352962293074805895248510699696029696 + (348437586779514700475067630180842053206482623665*sin(q1L))/2993155353253689176481146537402947624255349848014848 + (67682029681889335677290557259385*cos(q2L)*((1888752292310023*cos(q1L))/18014398509481984 - (5148155107303929*sin(q1L))/9007199254740992))/332306998946228968225951765070086144 + (9007199067919185*sin(q2L)*((5148155107303929*cos(q1L))/9007199254740992 + (1888752292310023*sin(q1L))/18014398509481984))/9007199254740992 + 103474418939599489499345508650025439853395886685/3064991081731777716716694054300618367237478244367204352) - ((7514214926474921*cos(q4L))/36893488147419103232 + (4503599440548691*sin(q4L))/4503599627370496)*((9007199067919185*sin(q3L)*((46370457884011341126541404977865*sin(q1L))/81129638414606681695789005144064 - (17012367886825063216155529491255*cos(q1L))/162259276829213363391578010288128 + 13770489658876653055167369550485/83076749736557242056487941267521536))/9007199254740992 - (7514214926474921*sin(q3L)*((16506520352940097956833727997725*cos(q2L))/20282409603651670423947251286016 + (7514214926474921*cos(q2L)*((1888752292310023*cos(q1L))/18014398509481984 - (5148155107303929*sin(q1L))/9007199254740992))/36893488147419103232 + sin(q2L)*((5148155107303929*cos(q1L))/9007199254740992 + (1888752292310023*sin(q1L))/18014398509481984)))/36893488147419103232 + cos(q3L)*((16506520352940097956833727997725*sin(q2L))/20282409603651670423947251286016 - cos(q2L)*((5148155107303929*cos(q1L))/9007199254740992 + (1888752292310023*sin(q1L))/18014398509481984) + (7514214926474921*sin(q2L)*((1888752292310023*cos(q1L))/18014398509481984 - (5148155107303929*sin(q1L))/9007199254740992))/36893488147419103232)) + (7514214926474921*sin(q4L)*((7514214926474921*cos(q3L)*((16506520352940097956833727997725*cos(q2L))/20282409603651670423947251286016 + (7514214926474921*cos(q2L)*((1888752292310023*cos(q1L))/18014398509481984 - (5148155107303929*sin(q1L))/9007199254740992))/36893488147419103232 + sin(q2L)*((5148155107303929*cos(q1L))/9007199254740992 + (1888752292310023*sin(q1L))/18014398509481984)))/36893488147419103232 - (9007199067919185*cos(q3L)*((46370457884011341126541404977865*sin(q1L))/81129638414606681695789005144064 - (17012367886825063216155529491255*cos(q1L))/162259276829213363391578010288128 + 13770489658876653055167369550485/83076749736557242056487941267521536))/9007199254740992 + sin(q3L)*((16506520352940097956833727997725*sin(q2L))/20282409603651670423947251286016 - cos(q2L)*((5148155107303929*cos(q1L))/9007199254740992 + (1888752292310023*sin(q1L))/18014398509481984) + (7514214926474921*sin(q2L)*((1888752292310023*cos(q1L))/18014398509481984 - (5148155107303929*sin(q1L))/9007199254740992))/36893488147419103232)))/36893488147419103232))/2451992865385422173373355243440494693789982595493763481600 - (202883803014822867*sin(q5L)*(((9007199067919185*cos(q4L))/9007199254740992 - (234819211581865*sin(q4L))/1152921504606846976)*((148677514737591106934298605035692608392163854125*cos(q2L))/182687704666362864775460604089535377456991567872 - (127834588709863499538908289888301307693646315855*cos(q1L))/5986310706507378352962293074805895248510699696029696 + (348437586779514700475067630180842053206482623665*sin(q1L))/2993155353253689176481146537402947624255349848014848 + (67682029681889335677290557259385*cos(q2L)*((1888752292310023*cos(q1L))/18014398509481984 - (5148155107303929*sin(q1L))/9007199254740992))/332306998946228968225951765070086144 + (9007199067919185*sin(q2L)*((5148155107303929*cos(q1L))/9007199254740992 + (1888752292310023*sin(q1L))/18014398509481984))/9007199254740992 + 103474418939599489499345508650025439853395886685/3064991081731777716716694054300618367237478244367204352) - ((7514214926474921*cos(q4L))/36893488147419103232 + (4503599440548691*sin(q4L))/4503599627370496)*((9007199067919185*sin(q3L)*((46370457884011341126541404977865*sin(q1L))/81129638414606681695789005144064 - (17012367886825063216155529491255*cos(q1L))/162259276829213363391578010288128 + 13770489658876653055167369550485/83076749736557242056487941267521536))/9007199254740992 - (7514214926474921*sin(q3L)*((16506520352940097956833727997725*cos(q2L))/20282409603651670423947251286016 + (7514214926474921*cos(q2L)*((1888752292310023*cos(q1L))/18014398509481984 - (5148155107303929*sin(q1L))/9007199254740992))/36893488147419103232 + sin(q2L)*((5148155107303929*cos(q1L))/9007199254740992 + (1888752292310023*sin(q1L))/18014398509481984)))/36893488147419103232 + cos(q3L)*((16506520352940097956833727997725*sin(q2L))/20282409603651670423947251286016 - cos(q2L)*((5148155107303929*cos(q1L))/9007199254740992 + (1888752292310023*sin(q1L))/18014398509481984) + (7514214926474921*sin(q2L)*((1888752292310023*cos(q1L))/18014398509481984 - (5148155107303929*sin(q1L))/9007199254740992))/36893488147419103232)) + (7514214926474921*sin(q4L)*((7514214926474921*cos(q3L)*((16506520352940097956833727997725*cos(q2L))/20282409603651670423947251286016 + (7514214926474921*cos(q2L)*((1888752292310023*cos(q1L))/18014398509481984 - (5148155107303929*sin(q1L))/9007199254740992))/36893488147419103232 + sin(q2L)*((5148155107303929*cos(q1L))/9007199254740992 + (1888752292310023*sin(q1L))/18014398509481984)))/36893488147419103232 - (9007199067919185*cos(q3L)*((46370457884011341126541404977865*sin(q1L))/81129638414606681695789005144064 - (17012367886825063216155529491255*cos(q1L))/162259276829213363391578010288128 + 13770489658876653055167369550485/83076749736557242056487941267521536))/9007199254740992 + sin(q3L)*((16506520352940097956833727997725*sin(q2L))/20282409603651670423947251286016 - cos(q2L)*((5148155107303929*cos(q1L))/9007199254740992 + (1888752292310023*sin(q1L))/18014398509481984) + (7514214926474921*sin(q2L)*((1888752292310023*cos(q1L))/18014398509481984 - (5148155107303929*sin(q1L))/9007199254740992))/36893488147419103232)))/36893488147419103232))/36893488147419103232000 + (608651409044468601*cos(q4L)*((7514214926474921*cos(q3L)*((16506520352940097956833727997725*cos(q2L))/20282409603651670423947251286016 + (7514214926474921*cos(q2L)*((1888752292310023*cos(q1L))/18014398509481984 - (5148155107303929*sin(q1L))/9007199254740992))/36893488147419103232 + sin(q2L)*((5148155107303929*cos(q1L))/9007199254740992 + (1888752292310023*sin(q1L))/18014398509481984)))/36893488147419103232 - (9007199067919185*cos(q3L)*((46370457884011341126541404977865*sin(q1L))/81129638414606681695789005144064 - (17012367886825063216155529491255*cos(q1L))/162259276829213363391578010288128 + 13770489658876653055167369550485/83076749736557242056487941267521536))/9007199254740992 + sin(q3L)*((16506520352940097956833727997725*sin(q2L))/20282409603651670423947251286016 - cos(q2L)*((5148155107303929*cos(q1L))/9007199254740992 + (1888752292310023*sin(q1L))/18014398509481984) + (7514214926474921*sin(q2L)*((1888752292310023*cos(q1L))/18014398509481984 - (5148155107303929*sin(q1L))/9007199254740992))/36893488147419103232)))/73786976294838206464000 - (610321541873521657855151997354401418608858870661075444886782706002880706727*sin(q4L)*((7514214926474921*cos(q3L)*((16506520352940097956833727997725*cos(q2L))/20282409603651670423947251286016 + (7514214926474921*cos(q2L)*((1888752292310023*cos(q1L))/18014398509481984 - (5148155107303929*sin(q1L))/9007199254740992))/36893488147419103232 + sin(q2L)*((5148155107303929*cos(q1L))/9007199254740992 + (1888752292310023*sin(q1L))/18014398509481984)))/36893488147419103232 - (9007199067919185*cos(q3L)*((46370457884011341126541404977865*sin(q1L))/81129638414606681695789005144064 - (17012367886825063216155529491255*cos(q1L))/162259276829213363391578010288128 + 13770489658876653055167369550485/83076749736557242056487941267521536))/9007199254740992 + sin(q3L)*((16506520352940097956833727997725*sin(q2L))/20282409603651670423947251286016 - cos(q2L)*((5148155107303929*cos(q1L))/9007199254740992 + (1888752292310023*sin(q1L))/18014398509481984) + (7514214926474921*sin(q2L)*((1888752292310023*cos(q1L))/18014398509481984 - (5148155107303929*sin(q1L))/9007199254740992))/36893488147419103232)))/11307821214581659709333104004754678501295896940003961331978279688272766566400000, (48638874966763599*cos(q5L)*((233003667623740560033643537092505706768317191960312467162596875*cos(q2L))/6901746346790563787434755862277025452451108972170386555162524223799296 - (200339157344278917575443724098432450908090682630030995291449625*cos(q1L))/226156424291633194186662080095093570025917938800079226639565593765455331328 + (546062636309760713610973115066597791006802105742542518556166375*sin(q1L))/113078212145816597093331040047546785012958969400039613319782796882727665664 - (81129635049124235038645691064225*cos(q3L)*((46370457884011341126541404977865*sin(q1L))/81129638414606681695789005144064 - (17012367886825063216155529491255*cos(q1L))/162259276829213363391578010288128 + 13770489658876653055167369550485/83076749736557242056487941267521536))/81129638414606681695789005144064 + (2115063383689692319117831580025*sin(q3L)*((46370457884011341126541404977865*sin(q1L))/81129638414606681695789005144064 - (17012367886825063216155529491255*cos(q1L))/162259276829213363391578010288128 + 13770489658876653055167369550485/83076749736557242056487941267521536))/10384593717069655257060992658440192 + (106069577339469832923929692356850887620017617375*cos(q2L)*((1888752292310023*cos(q1L))/18014398509481984 - (5148155107303929*sin(q1L))/9007199254740992))/12554203470773361527671578846415332832204710888928069025792 + (67682029681889335677290557259385*cos(q3L)*((16506520352940097956833727997725*cos(q2L))/20282409603651670423947251286016 + (7514214926474921*cos(q2L)*((1888752292310023*cos(q1L))/18014398509481984 - (5148155107303929*sin(q1L))/9007199254740992))/36893488147419103232 + sin(q2L)*((5148155107303929*cos(q1L))/9007199254740992 + (1888752292310023*sin(q1L))/18014398509481984)))/332306998946228968225951765070086144 + (14115856197532180673579726082375*sin(q2L)*((5148155107303929*cos(q1L))/9007199254740992 + (1888752292310023*sin(q1L))/18014398509481984))/340282366920938463463374607431768211456 - (1764482024691522628700660907665*sin(q3L)*((16506520352940097956833727997725*cos(q2L))/20282409603651670423947251286016 + (7514214926474921*cos(q2L)*((1888752292310023*cos(q1L))/18014398509481984 - (5148155107303929*sin(q1L))/9007199254740992))/36893488147419103232 + sin(q2L)*((5148155107303929*cos(q1L))/9007199254740992 + (1888752292310023*sin(q1L))/18014398509481984)))/42535295865117307932921825928971026432 + (234819211581865*cos(q3L)*((16506520352940097956833727997725*sin(q2L))/20282409603651670423947251286016 - cos(q2L)*((5148155107303929*cos(q1L))/9007199254740992 + (1888752292310023*sin(q1L))/18014398509481984) + (7514214926474921*sin(q2L)*((1888752292310023*cos(q1L))/18014398509481984 - (5148155107303929*sin(q1L))/9007199254740992))/36893488147419103232))/1152921504606846976 + (9007199067919185*sin(q3L)*((16506520352940097956833727997725*sin(q2L))/20282409603651670423947251286016 - cos(q2L)*((5148155107303929*cos(q1L))/9007199254740992 + (1888752292310023*sin(q1L))/18014398509481984) + (7514214926474921*sin(q2L)*((1888752292310023*cos(q1L))/18014398509481984 - (5148155107303929*sin(q1L))/9007199254740992))/36893488147419103232))/9007199254740992 + 162162510993777435611894002759555259653680159872115681607894875/115792089237316195423570985008687907853269984665640564039457584007913129639936))/1801439850948198400 - (202883803014822867*cos(q5L)*(((4503599440548691*cos(q4L))/4503599627370496 - (7514214926474921*sin(q4L))/36893488147419103232)*((9007199067919185*sin(q3L)*((46370457884011341126541404977865*sin(q1L))/81129638414606681695789005144064 - (17012367886825063216155529491255*cos(q1L))/162259276829213363391578010288128 + 13770489658876653055167369550485/83076749736557242056487941267521536))/9007199254740992 - (7514214926474921*sin(q3L)*((16506520352940097956833727997725*cos(q2L))/20282409603651670423947251286016 + (7514214926474921*cos(q2L)*((1888752292310023*cos(q1L))/18014398509481984 - (5148155107303929*sin(q1L))/9007199254740992))/36893488147419103232 + sin(q2L)*((5148155107303929*cos(q1L))/9007199254740992 + (1888752292310023*sin(q1L))/18014398509481984)))/36893488147419103232 + cos(q3L)*((16506520352940097956833727997725*sin(q2L))/20282409603651670423947251286016 - cos(q2L)*((5148155107303929*cos(q1L))/9007199254740992 + (1888752292310023*sin(q1L))/18014398509481984) + (7514214926474921*sin(q2L)*((1888752292310023*cos(q1L))/18014398509481984 - (5148155107303929*sin(q1L))/9007199254740992))/36893488147419103232)) + ((234819211581865*cos(q4L))/1152921504606846976 + (9007199067919185*sin(q4L))/9007199254740992)*((148677514737591106934298605035692608392163854125*cos(q2L))/182687704666362864775460604089535377456991567872 - (127834588709863499538908289888301307693646315855*cos(q1L))/5986310706507378352962293074805895248510699696029696 + (348437586779514700475067630180842053206482623665*sin(q1L))/2993155353253689176481146537402947624255349848014848 + (67682029681889335677290557259385*cos(q2L)*((1888752292310023*cos(q1L))/18014398509481984 - (5148155107303929*sin(q1L))/9007199254740992))/332306998946228968225951765070086144 + (9007199067919185*sin(q2L)*((5148155107303929*cos(q1L))/9007199254740992 + (1888752292310023*sin(q1L))/18014398509481984))/9007199254740992 + 103474418939599489499345508650025439853395886685/3064991081731777716716694054300618367237478244367204352) - (7514214926474921*cos(q4L)*((7514214926474921*cos(q3L)*((16506520352940097956833727997725*cos(q2L))/20282409603651670423947251286016 + (7514214926474921*cos(q2L)*((1888752292310023*cos(q1L))/18014398509481984 - (5148155107303929*sin(q1L))/9007199254740992))/36893488147419103232 + sin(q2L)*((5148155107303929*cos(q1L))/9007199254740992 + (1888752292310023*sin(q1L))/18014398509481984)))/36893488147419103232 - (9007199067919185*cos(q3L)*((46370457884011341126541404977865*sin(q1L))/81129638414606681695789005144064 - (17012367886825063216155529491255*cos(q1L))/162259276829213363391578010288128 + 13770489658876653055167369550485/83076749736557242056487941267521536))/9007199254740992 + sin(q3L)*((16506520352940097956833727997725*sin(q2L))/20282409603651670423947251286016 - cos(q2L)*((5148155107303929*cos(q1L))/9007199254740992 + (1888752292310023*sin(q1L))/18014398509481984) + (7514214926474921*sin(q2L)*((1888752292310023*cos(q1L))/18014398509481984 - (5148155107303929*sin(q1L))/9007199254740992))/36893488147419103232)))/36893488147419103232))/36893488147419103232000 + (170695144106365826517608855445768431563113584343*sin(q5L)*((233003667623740560033643537092505706768317191960312467162596875*cos(q2L))/6901746346790563787434755862277025452451108972170386555162524223799296 - (200339157344278917575443724098432450908090682630030995291449625*cos(q1L))/226156424291633194186662080095093570025917938800079226639565593765455331328 + (546062636309760713610973115066597791006802105742542518556166375*sin(q1L))/113078212145816597093331040047546785012958969400039613319782796882727665664 - (81129635049124235038645691064225*cos(q3L)*((46370457884011341126541404977865*sin(q1L))/81129638414606681695789005144064 - (17012367886825063216155529491255*cos(q1L))/162259276829213363391578010288128 + 13770489658876653055167369550485/83076749736557242056487941267521536))/81129638414606681695789005144064 + (2115063383689692319117831580025*sin(q3L)*((46370457884011341126541404977865*sin(q1L))/81129638414606681695789005144064 - (17012367886825063216155529491255*cos(q1L))/162259276829213363391578010288128 + 13770489658876653055167369550485/83076749736557242056487941267521536))/10384593717069655257060992658440192 + (106069577339469832923929692356850887620017617375*cos(q2L)*((1888752292310023*cos(q1L))/18014398509481984 - (5148155107303929*sin(q1L))/9007199254740992))/12554203470773361527671578846415332832204710888928069025792 + (67682029681889335677290557259385*cos(q3L)*((16506520352940097956833727997725*cos(q2L))/20282409603651670423947251286016 + (7514214926474921*cos(q2L)*((1888752292310023*cos(q1L))/18014398509481984 - (5148155107303929*sin(q1L))/9007199254740992))/36893488147419103232 + sin(q2L)*((5148155107303929*cos(q1L))/9007199254740992 + (1888752292310023*sin(q1L))/18014398509481984)))/332306998946228968225951765070086144 + (14115856197532180673579726082375*sin(q2L)*((5148155107303929*cos(q1L))/9007199254740992 + (1888752292310023*sin(q1L))/18014398509481984))/340282366920938463463374607431768211456 - (1764482024691522628700660907665*sin(q3L)*((16506520352940097956833727997725*cos(q2L))/20282409603651670423947251286016 + (7514214926474921*cos(q2L)*((1888752292310023*cos(q1L))/18014398509481984 - (5148155107303929*sin(q1L))/9007199254740992))/36893488147419103232 + sin(q2L)*((5148155107303929*cos(q1L))/9007199254740992 + (1888752292310023*sin(q1L))/18014398509481984)))/42535295865117307932921825928971026432 + (234819211581865*cos(q3L)*((16506520352940097956833727997725*sin(q2L))/20282409603651670423947251286016 - cos(q2L)*((5148155107303929*cos(q1L))/9007199254740992 + (1888752292310023*sin(q1L))/18014398509481984) + (7514214926474921*sin(q2L)*((1888752292310023*cos(q1L))/18014398509481984 - (5148155107303929*sin(q1L))/9007199254740992))/36893488147419103232))/1152921504606846976 + (9007199067919185*sin(q3L)*((16506520352940097956833727997725*sin(q2L))/20282409603651670423947251286016 - cos(q2L)*((5148155107303929*cos(q1L))/9007199254740992 + (1888752292310023*sin(q1L))/18014398509481984) + (7514214926474921*sin(q2L)*((1888752292310023*cos(q1L))/18014398509481984 - (5148155107303929*sin(q1L))/9007199254740992))/36893488147419103232))/9007199254740992 + 162162510993777435611894002759555259653680159872115681607894875/115792089237316195423570985008687907853269984665640564039457584007913129639936))/119726214130147567059245861496117904970213993920593920 - (712008244765680093343103025701132101054572137019*sin(q5L)*(((4503599440548691*cos(q4L))/4503599627370496 - (7514214926474921*sin(q4L))/36893488147419103232)*((9007199067919185*sin(q3L)*((46370457884011341126541404977865*sin(q1L))/81129638414606681695789005144064 - (17012367886825063216155529491255*cos(q1L))/162259276829213363391578010288128 + 13770489658876653055167369550485/83076749736557242056487941267521536))/9007199254740992 - (7514214926474921*sin(q3L)*((16506520352940097956833727997725*cos(q2L))/20282409603651670423947251286016 + (7514214926474921*cos(q2L)*((1888752292310023*cos(q1L))/18014398509481984 - (5148155107303929*sin(q1L))/9007199254740992))/36893488147419103232 + sin(q2L)*((5148155107303929*cos(q1L))/9007199254740992 + (1888752292310023*sin(q1L))/18014398509481984)))/36893488147419103232 + cos(q3L)*((16506520352940097956833727997725*sin(q2L))/20282409603651670423947251286016 - cos(q2L)*((5148155107303929*cos(q1L))/9007199254740992 + (1888752292310023*sin(q1L))/18014398509481984) + (7514214926474921*sin(q2L)*((1888752292310023*cos(q1L))/18014398509481984 - (5148155107303929*sin(q1L))/9007199254740992))/36893488147419103232)) + ((234819211581865*cos(q4L))/1152921504606846976 + (9007199067919185*sin(q4L))/9007199254740992)*((148677514737591106934298605035692608392163854125*cos(q2L))/182687704666362864775460604089535377456991567872 - (127834588709863499538908289888301307693646315855*cos(q1L))/5986310706507378352962293074805895248510699696029696 + (348437586779514700475067630180842053206482623665*sin(q1L))/2993155353253689176481146537402947624255349848014848 + (67682029681889335677290557259385*cos(q2L)*((1888752292310023*cos(q1L))/18014398509481984 - (5148155107303929*sin(q1L))/9007199254740992))/332306998946228968225951765070086144 + (9007199067919185*sin(q2L)*((5148155107303929*cos(q1L))/9007199254740992 + (1888752292310023*sin(q1L))/18014398509481984))/9007199254740992 + 103474418939599489499345508650025439853395886685/3064991081731777716716694054300618367237478244367204352) - (7514214926474921*cos(q4L)*((7514214926474921*cos(q3L)*((16506520352940097956833727997725*cos(q2L))/20282409603651670423947251286016 + (7514214926474921*cos(q2L)*((1888752292310023*cos(q1L))/18014398509481984 - (5148155107303929*sin(q1L))/9007199254740992))/36893488147419103232 + sin(q2L)*((5148155107303929*cos(q1L))/9007199254740992 + (1888752292310023*sin(q1L))/18014398509481984)))/36893488147419103232 - (9007199067919185*cos(q3L)*((46370457884011341126541404977865*sin(q1L))/81129638414606681695789005144064 - (17012367886825063216155529491255*cos(q1L))/162259276829213363391578010288128 + 13770489658876653055167369550485/83076749736557242056487941267521536))/9007199254740992 + sin(q3L)*((16506520352940097956833727997725*sin(q2L))/20282409603651670423947251286016 - cos(q2L)*((5148155107303929*cos(q1L))/9007199254740992 + (1888752292310023*sin(q1L))/18014398509481984) + (7514214926474921*sin(q2L)*((1888752292310023*cos(q1L))/18014398509481984 - (5148155107303929*sin(q1L))/9007199254740992))/36893488147419103232)))/36893488147419103232))/2451992865385422173373355243440494693789982595493763481600 - (94754841554645069948206780163139*cos(q5L)*(((9007199067919185*cos(q4L))/9007199254740992 - (234819211581865*sin(q4L))/1152921504606846976)*((148677514737591106934298605035692608392163854125*cos(q2L))/182687704666362864775460604089535377456991567872 - (127834588709863499538908289888301307693646315855*cos(q1L))/5986310706507378352962293074805895248510699696029696 + (348437586779514700475067630180842053206482623665*sin(q1L))/2993155353253689176481146537402947624255349848014848 + (67682029681889335677290557259385*cos(q2L)*((1888752292310023*cos(q1L))/18014398509481984 - (5148155107303929*sin(q1L))/9007199254740992))/332306998946228968225951765070086144 + (9007199067919185*sin(q2L)*((5148155107303929*cos(q1L))/9007199254740992 + (1888752292310023*sin(q1L))/18014398509481984))/9007199254740992 + 103474418939599489499345508650025439853395886685/3064991081731777716716694054300618367237478244367204352) - ((7514214926474921*cos(q4L))/36893488147419103232 + (4503599440548691*sin(q4L))/4503599627370496)*((9007199067919185*sin(q3L)*((46370457884011341126541404977865*sin(q1L))/81129638414606681695789005144064 - (17012367886825063216155529491255*cos(q1L))/162259276829213363391578010288128 + 13770489658876653055167369550485/83076749736557242056487941267521536))/9007199254740992 - (7514214926474921*sin(q3L)*((16506520352940097956833727997725*cos(q2L))/20282409603651670423947251286016 + (7514214926474921*cos(q2L)*((1888752292310023*cos(q1L))/18014398509481984 - (5148155107303929*sin(q1L))/9007199254740992))/36893488147419103232 + sin(q2L)*((5148155107303929*cos(q1L))/9007199254740992 + (1888752292310023*sin(q1L))/18014398509481984)))/36893488147419103232 + cos(q3L)*((16506520352940097956833727997725*sin(q2L))/20282409603651670423947251286016 - cos(q2L)*((5148155107303929*cos(q1L))/9007199254740992 + (1888752292310023*sin(q1L))/18014398509481984) + (7514214926474921*sin(q2L)*((1888752292310023*cos(q1L))/18014398509481984 - (5148155107303929*sin(q1L))/9007199254740992))/36893488147419103232)) + (7514214926474921*sin(q4L)*((7514214926474921*cos(q3L)*((16506520352940097956833727997725*cos(q2L))/20282409603651670423947251286016 + (7514214926474921*cos(q2L)*((1888752292310023*cos(q1L))/18014398509481984 - (5148155107303929*sin(q1L))/9007199254740992))/36893488147419103232 + sin(q2L)*((5148155107303929*cos(q1L))/9007199254740992 + (1888752292310023*sin(q1L))/18014398509481984)))/36893488147419103232 - (9007199067919185*cos(q3L)*((46370457884011341126541404977865*sin(q1L))/81129638414606681695789005144064 - (17012367886825063216155529491255*cos(q1L))/162259276829213363391578010288128 + 13770489658876653055167369550485/83076749736557242056487941267521536))/9007199254740992 + sin(q3L)*((16506520352940097956833727997725*sin(q2L))/20282409603651670423947251286016 - cos(q2L)*((5148155107303929*cos(q1L))/9007199254740992 + (1888752292310023*sin(q1L))/18014398509481984) + (7514214926474921*sin(q2L)*((1888752292310023*cos(q1L))/18014398509481984 - (5148155107303929*sin(q1L))/9007199254740992))/36893488147419103232)))/36893488147419103232))/66461399789245793645190353014017228800 + (27*sin(q5L)*(((9007199067919185*cos(q4L))/9007199254740992 - (234819211581865*sin(q4L))/1152921504606846976)*((148677514737591106934298605035692608392163854125*cos(q2L))/182687704666362864775460604089535377456991567872 - (127834588709863499538908289888301307693646315855*cos(q1L))/5986310706507378352962293074805895248510699696029696 + (348437586779514700475067630180842053206482623665*sin(q1L))/2993155353253689176481146537402947624255349848014848 + (67682029681889335677290557259385*cos(q2L)*((1888752292310023*cos(q1L))/18014398509481984 - (5148155107303929*sin(q1L))/9007199254740992))/332306998946228968225951765070086144 + (9007199067919185*sin(q2L)*((5148155107303929*cos(q1L))/9007199254740992 + (1888752292310023*sin(q1L))/18014398509481984))/9007199254740992 + 103474418939599489499345508650025439853395886685/3064991081731777716716694054300618367237478244367204352) - ((7514214926474921*cos(q4L))/36893488147419103232 + (4503599440548691*sin(q4L))/4503599627370496)*((9007199067919185*sin(q3L)*((46370457884011341126541404977865*sin(q1L))/81129638414606681695789005144064 - (17012367886825063216155529491255*cos(q1L))/162259276829213363391578010288128 + 13770489658876653055167369550485/83076749736557242056487941267521536))/9007199254740992 - (7514214926474921*sin(q3L)*((16506520352940097956833727997725*cos(q2L))/20282409603651670423947251286016 + (7514214926474921*cos(q2L)*((1888752292310023*cos(q1L))/18014398509481984 - (5148155107303929*sin(q1L))/9007199254740992))/36893488147419103232 + sin(q2L)*((5148155107303929*cos(q1L))/9007199254740992 + (1888752292310023*sin(q1L))/18014398509481984)))/36893488147419103232 + cos(q3L)*((16506520352940097956833727997725*sin(q2L))/20282409603651670423947251286016 - cos(q2L)*((5148155107303929*cos(q1L))/9007199254740992 + (1888752292310023*sin(q1L))/18014398509481984) + (7514214926474921*sin(q2L)*((1888752292310023*cos(q1L))/18014398509481984 - (5148155107303929*sin(q1L))/9007199254740992))/36893488147419103232)) + (7514214926474921*sin(q4L)*((7514214926474921*cos(q3L)*((16506520352940097956833727997725*cos(q2L))/20282409603651670423947251286016 + (7514214926474921*cos(q2L)*((1888752292310023*cos(q1L))/18014398509481984 - (5148155107303929*sin(q1L))/9007199254740992))/36893488147419103232 + sin(q2L)*((5148155107303929*cos(q1L))/9007199254740992 + (1888752292310023*sin(q1L))/18014398509481984)))/36893488147419103232 - (9007199067919185*cos(q3L)*((46370457884011341126541404977865*sin(q1L))/81129638414606681695789005144064 - (17012367886825063216155529491255*cos(q1L))/162259276829213363391578010288128 + 13770489658876653055167369550485/83076749736557242056487941267521536))/9007199254740992 + sin(q3L)*((16506520352940097956833727997725*sin(q2L))/20282409603651670423947251286016 - cos(q2L)*((5148155107303929*cos(q1L))/9007199254740992 + (1888752292310023*sin(q1L))/18014398509481984) + (7514214926474921*sin(q2L)*((1888752292310023*cos(q1L))/18014398509481984 - (5148155107303929*sin(q1L))/9007199254740992))/36893488147419103232)))/36893488147419103232))/1000 - (27*cos(q6L)*((9007199067919185*cos(q5L)*((233003667623740560033643537092505706768317191960312467162596875*cos(q2L))/6901746346790563787434755862277025452451108972170386555162524223799296 - (200339157344278917575443724098432450908090682630030995291449625*cos(q1L))/226156424291633194186662080095093570025917938800079226639565593765455331328 + (546062636309760713610973115066597791006802105742542518556166375*sin(q1L))/113078212145816597093331040047546785012958969400039613319782796882727665664 - (81129635049124235038645691064225*cos(q3L)*((46370457884011341126541404977865*sin(q1L))/81129638414606681695789005144064 - (17012367886825063216155529491255*cos(q1L))/162259276829213363391578010288128 + 13770489658876653055167369550485/83076749736557242056487941267521536))/81129638414606681695789005144064 + (2115063383689692319117831580025*sin(q3L)*((46370457884011341126541404977865*sin(q1L))/81129638414606681695789005144064 - (17012367886825063216155529491255*cos(q1L))/162259276829213363391578010288128 + 13770489658876653055167369550485/83076749736557242056487941267521536))/10384593717069655257060992658440192 + (106069577339469832923929692356850887620017617375*cos(q2L)*((1888752292310023*cos(q1L))/18014398509481984 - (5148155107303929*sin(q1L))/9007199254740992))/12554203470773361527671578846415332832204710888928069025792 + (67682029681889335677290557259385*cos(q3L)*((16506520352940097956833727997725*cos(q2L))/20282409603651670423947251286016 + (7514214926474921*cos(q2L)*((1888752292310023*cos(q1L))/18014398509481984 - (5148155107303929*sin(q1L))/9007199254740992))/36893488147419103232 + sin(q2L)*((5148155107303929*cos(q1L))/9007199254740992 + (1888752292310023*sin(q1L))/18014398509481984)))/332306998946228968225951765070086144 + (14115856197532180673579726082375*sin(q2L)*((5148155107303929*cos(q1L))/9007199254740992 + (1888752292310023*sin(q1L))/18014398509481984))/340282366920938463463374607431768211456 - (1764482024691522628700660907665*sin(q3L)*((16506520352940097956833727997725*cos(q2L))/20282409603651670423947251286016 + (7514214926474921*cos(q2L)*((1888752292310023*cos(q1L))/18014398509481984 - (5148155107303929*sin(q1L))/9007199254740992))/36893488147419103232 + sin(q2L)*((5148155107303929*cos(q1L))/9007199254740992 + (1888752292310023*sin(q1L))/18014398509481984)))/42535295865117307932921825928971026432 + (234819211581865*cos(q3L)*((16506520352940097956833727997725*sin(q2L))/20282409603651670423947251286016 - cos(q2L)*((5148155107303929*cos(q1L))/9007199254740992 + (1888752292310023*sin(q1L))/18014398509481984) + (7514214926474921*sin(q2L)*((1888752292310023*cos(q1L))/18014398509481984 - (5148155107303929*sin(q1L))/9007199254740992))/36893488147419103232))/1152921504606846976 + (9007199067919185*sin(q3L)*((16506520352940097956833727997725*sin(q2L))/20282409603651670423947251286016 - cos(q2L)*((5148155107303929*cos(q1L))/9007199254740992 + (1888752292310023*sin(q1L))/18014398509481984) + (7514214926474921*sin(q2L)*((1888752292310023*cos(q1L))/18014398509481984 - (5148155107303929*sin(q1L))/9007199254740992))/36893488147419103232))/9007199254740992 + 162162510993777435611894002759555259653680159872115681607894875/115792089237316195423570985008687907853269984665640564039457584007913129639936))/9007199254740992 - (7514214926474921*cos(q5L)*(((4503599440548691*cos(q4L))/4503599627370496 - (7514214926474921*sin(q4L))/36893488147419103232)*((9007199067919185*sin(q3L)*((46370457884011341126541404977865*sin(q1L))/81129638414606681695789005144064 - (17012367886825063216155529491255*cos(q1L))/162259276829213363391578010288128 + 13770489658876653055167369550485/83076749736557242056487941267521536))/9007199254740992 - (7514214926474921*sin(q3L)*((16506520352940097956833727997725*cos(q2L))/20282409603651670423947251286016 + (7514214926474921*cos(q2L)*((1888752292310023*cos(q1L))/18014398509481984 - (5148155107303929*sin(q1L))/9007199254740992))/36893488147419103232 + sin(q2L)*((5148155107303929*cos(q1L))/9007199254740992 + (1888752292310023*sin(q1L))/18014398509481984)))/36893488147419103232 + cos(q3L)*((16506520352940097956833727997725*sin(q2L))/20282409603651670423947251286016 - cos(q2L)*((5148155107303929*cos(q1L))/9007199254740992 + (1888752292310023*sin(q1L))/18014398509481984) + (7514214926474921*sin(q2L)*((1888752292310023*cos(q1L))/18014398509481984 - (5148155107303929*sin(q1L))/9007199254740992))/36893488147419103232)) + ((234819211581865*cos(q4L))/1152921504606846976 + (9007199067919185*sin(q4L))/9007199254740992)*((148677514737591106934298605035692608392163854125*cos(q2L))/182687704666362864775460604089535377456991567872 - (127834588709863499538908289888301307693646315855*cos(q1L))/5986310706507378352962293074805895248510699696029696 + (348437586779514700475067630180842053206482623665*sin(q1L))/2993155353253689176481146537402947624255349848014848 + (67682029681889335677290557259385*cos(q2L)*((1888752292310023*cos(q1L))/18014398509481984 - (5148155107303929*sin(q1L))/9007199254740992))/332306998946228968225951765070086144 + (9007199067919185*sin(q2L)*((5148155107303929*cos(q1L))/9007199254740992 + (1888752292310023*sin(q1L))/18014398509481984))/9007199254740992 + 103474418939599489499345508650025439853395886685/3064991081731777716716694054300618367237478244367204352) - (7514214926474921*cos(q4L)*((7514214926474921*cos(q3L)*((16506520352940097956833727997725*cos(q2L))/20282409603651670423947251286016 + (7514214926474921*cos(q2L)*((1888752292310023*cos(q1L))/18014398509481984 - (5148155107303929*sin(q1L))/9007199254740992))/36893488147419103232 + sin(q2L)*((5148155107303929*cos(q1L))/9007199254740992 + (1888752292310023*sin(q1L))/18014398509481984)))/36893488147419103232 - (9007199067919185*cos(q3L)*((46370457884011341126541404977865*sin(q1L))/81129638414606681695789005144064 - (17012367886825063216155529491255*cos(q1L))/162259276829213363391578010288128 + 13770489658876653055167369550485/83076749736557242056487941267521536))/9007199254740992 + sin(q3L)*((16506520352940097956833727997725*sin(q2L))/20282409603651670423947251286016 - cos(q2L)*((5148155107303929*cos(q1L))/9007199254740992 + (1888752292310023*sin(q1L))/18014398509481984) + (7514214926474921*sin(q2L)*((1888752292310023*cos(q1L))/18014398509481984 - (5148155107303929*sin(q1L))/9007199254740992))/36893488147419103232)))/36893488147419103232))/36893488147419103232 + sin(q5L)*(((9007199067919185*cos(q4L))/9007199254740992 - (234819211581865*sin(q4L))/1152921504606846976)*((148677514737591106934298605035692608392163854125*cos(q2L))/182687704666362864775460604089535377456991567872 - (127834588709863499538908289888301307693646315855*cos(q1L))/5986310706507378352962293074805895248510699696029696 + (348437586779514700475067630180842053206482623665*sin(q1L))/2993155353253689176481146537402947624255349848014848 + (67682029681889335677290557259385*cos(q2L)*((1888752292310023*cos(q1L))/18014398509481984 - (5148155107303929*sin(q1L))/9007199254740992))/332306998946228968225951765070086144 + (9007199067919185*sin(q2L)*((5148155107303929*cos(q1L))/9007199254740992 + (1888752292310023*sin(q1L))/18014398509481984))/9007199254740992 + 103474418939599489499345508650025439853395886685/3064991081731777716716694054300618367237478244367204352) - ((7514214926474921*cos(q4L))/36893488147419103232 + (4503599440548691*sin(q4L))/4503599627370496)*((9007199067919185*sin(q3L)*((46370457884011341126541404977865*sin(q1L))/81129638414606681695789005144064 - (17012367886825063216155529491255*cos(q1L))/162259276829213363391578010288128 + 13770489658876653055167369550485/83076749736557242056487941267521536))/9007199254740992 - (7514214926474921*sin(q3L)*((16506520352940097956833727997725*cos(q2L))/20282409603651670423947251286016 + (7514214926474921*cos(q2L)*((1888752292310023*cos(q1L))/18014398509481984 - (5148155107303929*sin(q1L))/9007199254740992))/36893488147419103232 + sin(q2L)*((5148155107303929*cos(q1L))/9007199254740992 + (1888752292310023*sin(q1L))/18014398509481984)))/36893488147419103232 + cos(q3L)*((16506520352940097956833727997725*sin(q2L))/20282409603651670423947251286016 - cos(q2L)*((5148155107303929*cos(q1L))/9007199254740992 + (1888752292310023*sin(q1L))/18014398509481984) + (7514214926474921*sin(q2L)*((1888752292310023*cos(q1L))/18014398509481984 - (5148155107303929*sin(q1L))/9007199254740992))/36893488147419103232)) + (7514214926474921*sin(q4L)*((7514214926474921*cos(q3L)*((16506520352940097956833727997725*cos(q2L))/20282409603651670423947251286016 + (7514214926474921*cos(q2L)*((1888752292310023*cos(q1L))/18014398509481984 - (5148155107303929*sin(q1L))/9007199254740992))/36893488147419103232 + sin(q2L)*((5148155107303929*cos(q1L))/9007199254740992 + (1888752292310023*sin(q1L))/18014398509481984)))/36893488147419103232 - (9007199067919185*cos(q3L)*((46370457884011341126541404977865*sin(q1L))/81129638414606681695789005144064 - (17012367886825063216155529491255*cos(q1L))/162259276829213363391578010288128 + 13770489658876653055167369550485/83076749736557242056487941267521536))/9007199254740992 + sin(q3L)*((16506520352940097956833727997725*sin(q2L))/20282409603651670423947251286016 - cos(q2L)*((5148155107303929*cos(q1L))/9007199254740992 + (1888752292310023*sin(q1L))/18014398509481984) + (7514214926474921*sin(q2L)*((1888752292310023*cos(q1L))/18014398509481984 - (5148155107303929*sin(q1L))/9007199254740992))/36893488147419103232)))/36893488147419103232)))/1000 + (2436553109258773196144549622003023*cos(q6L)*((7514214926474921*sin(q5L)*(((4503599440548691*cos(q4L))/4503599627370496 - (7514214926474921*sin(q4L))/36893488147419103232)*((9007199067919185*sin(q3L)*((46370457884011341126541404977865*sin(q1L))/81129638414606681695789005144064 - (17012367886825063216155529491255*cos(q1L))/162259276829213363391578010288128 + 13770489658876653055167369550485/83076749736557242056487941267521536))/9007199254740992 - (7514214926474921*sin(q3L)*((16506520352940097956833727997725*cos(q2L))/20282409603651670423947251286016 + (7514214926474921*cos(q2L)*((1888752292310023*cos(q1L))/18014398509481984 - (5148155107303929*sin(q1L))/9007199254740992))/36893488147419103232 + sin(q2L)*((5148155107303929*cos(q1L))/9007199254740992 + (1888752292310023*sin(q1L))/18014398509481984)))/36893488147419103232 + cos(q3L)*((16506520352940097956833727997725*sin(q2L))/20282409603651670423947251286016 - cos(q2L)*((5148155107303929*cos(q1L))/9007199254740992 + (1888752292310023*sin(q1L))/18014398509481984) + (7514214926474921*sin(q2L)*((1888752292310023*cos(q1L))/18014398509481984 - (5148155107303929*sin(q1L))/9007199254740992))/36893488147419103232)) + ((234819211581865*cos(q4L))/1152921504606846976 + (9007199067919185*sin(q4L))/9007199254740992)*((148677514737591106934298605035692608392163854125*cos(q2L))/182687704666362864775460604089535377456991567872 - (127834588709863499538908289888301307693646315855*cos(q1L))/5986310706507378352962293074805895248510699696029696 + (348437586779514700475067630180842053206482623665*sin(q1L))/2993155353253689176481146537402947624255349848014848 + (67682029681889335677290557259385*cos(q2L)*((1888752292310023*cos(q1L))/18014398509481984 - (5148155107303929*sin(q1L))/9007199254740992))/332306998946228968225951765070086144 + (9007199067919185*sin(q2L)*((5148155107303929*cos(q1L))/9007199254740992 + (1888752292310023*sin(q1L))/18014398509481984))/9007199254740992 + 103474418939599489499345508650025439853395886685/3064991081731777716716694054300618367237478244367204352) - (7514214926474921*cos(q4L)*((7514214926474921*cos(q3L)*((16506520352940097956833727997725*cos(q2L))/20282409603651670423947251286016 + (7514214926474921*cos(q2L)*((1888752292310023*cos(q1L))/18014398509481984 - (5148155107303929*sin(q1L))/9007199254740992))/36893488147419103232 + sin(q2L)*((5148155107303929*cos(q1L))/9007199254740992 + (1888752292310023*sin(q1L))/18014398509481984)))/36893488147419103232 - (9007199067919185*cos(q3L)*((46370457884011341126541404977865*sin(q1L))/81129638414606681695789005144064 - (17012367886825063216155529491255*cos(q1L))/162259276829213363391578010288128 + 13770489658876653055167369550485/83076749736557242056487941267521536))/9007199254740992 + sin(q3L)*((16506520352940097956833727997725*sin(q2L))/20282409603651670423947251286016 - cos(q2L)*((5148155107303929*cos(q1L))/9007199254740992 + (1888752292310023*sin(q1L))/18014398509481984) + (7514214926474921*sin(q2L)*((1888752292310023*cos(q1L))/18014398509481984 - (5148155107303929*sin(q1L))/9007199254740992))/36893488147419103232)))/36893488147419103232))/36893488147419103232 - (9007199067919185*sin(q5L)*((233003667623740560033643537092505706768317191960312467162596875*cos(q2L))/6901746346790563787434755862277025452451108972170386555162524223799296 - (200339157344278917575443724098432450908090682630030995291449625*cos(q1L))/226156424291633194186662080095093570025917938800079226639565593765455331328 + (546062636309760713610973115066597791006802105742542518556166375*sin(q1L))/113078212145816597093331040047546785012958969400039613319782796882727665664 - (81129635049124235038645691064225*cos(q3L)*((46370457884011341126541404977865*sin(q1L))/81129638414606681695789005144064 - (17012367886825063216155529491255*cos(q1L))/162259276829213363391578010288128 + 13770489658876653055167369550485/83076749736557242056487941267521536))/81129638414606681695789005144064 + (2115063383689692319117831580025*sin(q3L)*((46370457884011341126541404977865*sin(q1L))/81129638414606681695789005144064 - (17012367886825063216155529491255*cos(q1L))/162259276829213363391578010288128 + 13770489658876653055167369550485/83076749736557242056487941267521536))/10384593717069655257060992658440192 + (106069577339469832923929692356850887620017617375*cos(q2L)*((1888752292310023*cos(q1L))/18014398509481984 - (5148155107303929*sin(q1L))/9007199254740992))/12554203470773361527671578846415332832204710888928069025792 + (67682029681889335677290557259385*cos(q3L)*((16506520352940097956833727997725*cos(q2L))/20282409603651670423947251286016 + (7514214926474921*cos(q2L)*((1888752292310023*cos(q1L))/18014398509481984 - (5148155107303929*sin(q1L))/9007199254740992))/36893488147419103232 + sin(q2L)*((5148155107303929*cos(q1L))/9007199254740992 + (1888752292310023*sin(q1L))/18014398509481984)))/332306998946228968225951765070086144 + (14115856197532180673579726082375*sin(q2L)*((5148155107303929*cos(q1L))/9007199254740992 + (1888752292310023*sin(q1L))/18014398509481984))/340282366920938463463374607431768211456 - (1764482024691522628700660907665*sin(q3L)*((16506520352940097956833727997725*cos(q2L))/20282409603651670423947251286016 + (7514214926474921*cos(q2L)*((1888752292310023*cos(q1L))/18014398509481984 - (5148155107303929*sin(q1L))/9007199254740992))/36893488147419103232 + sin(q2L)*((5148155107303929*cos(q1L))/9007199254740992 + (1888752292310023*sin(q1L))/18014398509481984)))/42535295865117307932921825928971026432 + (234819211581865*cos(q3L)*((16506520352940097956833727997725*sin(q2L))/20282409603651670423947251286016 - cos(q2L)*((5148155107303929*cos(q1L))/9007199254740992 + (1888752292310023*sin(q1L))/18014398509481984) + (7514214926474921*sin(q2L)*((1888752292310023*cos(q1L))/18014398509481984 - (5148155107303929*sin(q1L))/9007199254740992))/36893488147419103232))/1152921504606846976 + (9007199067919185*sin(q3L)*((16506520352940097956833727997725*sin(q2L))/20282409603651670423947251286016 - cos(q2L)*((5148155107303929*cos(q1L))/9007199254740992 + (1888752292310023*sin(q1L))/18014398509481984) + (7514214926474921*sin(q2L)*((1888752292310023*cos(q1L))/18014398509481984 - (5148155107303929*sin(q1L))/9007199254740992))/36893488147419103232))/9007199254740992 + 162162510993777435611894002759555259653680159872115681607894875/115792089237316195423570985008687907853269984665640564039457584007913129639936))/9007199254740992 + cos(q5L)*(((9007199067919185*cos(q4L))/9007199254740992 - (234819211581865*sin(q4L))/1152921504606846976)*((148677514737591106934298605035692608392163854125*cos(q2L))/182687704666362864775460604089535377456991567872 - (127834588709863499538908289888301307693646315855*cos(q1L))/5986310706507378352962293074805895248510699696029696 + (348437586779514700475067630180842053206482623665*sin(q1L))/2993155353253689176481146537402947624255349848014848 + (67682029681889335677290557259385*cos(q2L)*((1888752292310023*cos(q1L))/18014398509481984 - (5148155107303929*sin(q1L))/9007199254740992))/332306998946228968225951765070086144 + (9007199067919185*sin(q2L)*((5148155107303929*cos(q1L))/9007199254740992 + (1888752292310023*sin(q1L))/18014398509481984))/9007199254740992 + 103474418939599489499345508650025439853395886685/3064991081731777716716694054300618367237478244367204352) - ((7514214926474921*cos(q4L))/36893488147419103232 + (4503599440548691*sin(q4L))/4503599627370496)*((9007199067919185*sin(q3L)*((46370457884011341126541404977865*sin(q1L))/81129638414606681695789005144064 - (17012367886825063216155529491255*cos(q1L))/162259276829213363391578010288128 + 13770489658876653055167369550485/83076749736557242056487941267521536))/9007199254740992 - (7514214926474921*sin(q3L)*((16506520352940097956833727997725*cos(q2L))/20282409603651670423947251286016 + (7514214926474921*cos(q2L)*((1888752292310023*cos(q1L))/18014398509481984 - (5148155107303929*sin(q1L))/9007199254740992))/36893488147419103232 + sin(q2L)*((5148155107303929*cos(q1L))/9007199254740992 + (1888752292310023*sin(q1L))/18014398509481984)))/36893488147419103232 + cos(q3L)*((16506520352940097956833727997725*sin(q2L))/20282409603651670423947251286016 - cos(q2L)*((5148155107303929*cos(q1L))/9007199254740992 + (1888752292310023*sin(q1L))/18014398509481984) + (7514214926474921*sin(q2L)*((1888752292310023*cos(q1L))/18014398509481984 - (5148155107303929*sin(q1L))/9007199254740992))/36893488147419103232)) + (7514214926474921*sin(q4L)*((7514214926474921*cos(q3L)*((16506520352940097956833727997725*cos(q2L))/20282409603651670423947251286016 + (7514214926474921*cos(q2L)*((1888752292310023*cos(q1L))/18014398509481984 - (5148155107303929*sin(q1L))/9007199254740992))/36893488147419103232 + sin(q2L)*((5148155107303929*cos(q1L))/9007199254740992 + (1888752292310023*sin(q1L))/18014398509481984)))/36893488147419103232 - (9007199067919185*cos(q3L)*((46370457884011341126541404977865*sin(q1L))/81129638414606681695789005144064 - (17012367886825063216155529491255*cos(q1L))/162259276829213363391578010288128 + 13770489658876653055167369550485/83076749736557242056487941267521536))/9007199254740992 + sin(q3L)*((16506520352940097956833727997725*sin(q2L))/20282409603651670423947251286016 - cos(q2L)*((5148155107303929*cos(q1L))/9007199254740992 + (1888752292310023*sin(q1L))/18014398509481984) + (7514214926474921*sin(q2L)*((1888752292310023*cos(q1L))/18014398509481984 - (5148155107303929*sin(q1L))/9007199254740992))/36893488147419103232)))/36893488147419103232)))/332306998946228968225951765070086144000 + (324259171862923063*sin(q6L)*((9007199067919185*cos(q5L)*((233003667623740560033643537092505706768317191960312467162596875*cos(q2L))/6901746346790563787434755862277025452451108972170386555162524223799296 - (200339157344278917575443724098432450908090682630030995291449625*cos(q1L))/226156424291633194186662080095093570025917938800079226639565593765455331328 + (546062636309760713610973115066597791006802105742542518556166375*sin(q1L))/113078212145816597093331040047546785012958969400039613319782796882727665664 - (81129635049124235038645691064225*cos(q3L)*((46370457884011341126541404977865*sin(q1L))/81129638414606681695789005144064 - (17012367886825063216155529491255*cos(q1L))/162259276829213363391578010288128 + 13770489658876653055167369550485/83076749736557242056487941267521536))/81129638414606681695789005144064 + (2115063383689692319117831580025*sin(q3L)*((46370457884011341126541404977865*sin(q1L))/81129638414606681695789005144064 - (17012367886825063216155529491255*cos(q1L))/162259276829213363391578010288128 + 13770489658876653055167369550485/83076749736557242056487941267521536))/10384593717069655257060992658440192 + (106069577339469832923929692356850887620017617375*cos(q2L)*((1888752292310023*cos(q1L))/18014398509481984 - (5148155107303929*sin(q1L))/9007199254740992))/12554203470773361527671578846415332832204710888928069025792 + (67682029681889335677290557259385*cos(q3L)*((16506520352940097956833727997725*cos(q2L))/20282409603651670423947251286016 + (7514214926474921*cos(q2L)*((1888752292310023*cos(q1L))/18014398509481984 - (5148155107303929*sin(q1L))/9007199254740992))/36893488147419103232 + sin(q2L)*((5148155107303929*cos(q1L))/9007199254740992 + (1888752292310023*sin(q1L))/18014398509481984)))/332306998946228968225951765070086144 + (14115856197532180673579726082375*sin(q2L)*((5148155107303929*cos(q1L))/9007199254740992 + (1888752292310023*sin(q1L))/18014398509481984))/340282366920938463463374607431768211456 - (1764482024691522628700660907665*sin(q3L)*((16506520352940097956833727997725*cos(q2L))/20282409603651670423947251286016 + (7514214926474921*cos(q2L)*((1888752292310023*cos(q1L))/18014398509481984 - (5148155107303929*sin(q1L))/9007199254740992))/36893488147419103232 + sin(q2L)*((5148155107303929*cos(q1L))/9007199254740992 + (1888752292310023*sin(q1L))/18014398509481984)))/42535295865117307932921825928971026432 + (234819211581865*cos(q3L)*((16506520352940097956833727997725*sin(q2L))/20282409603651670423947251286016 - cos(q2L)*((5148155107303929*cos(q1L))/9007199254740992 + (1888752292310023*sin(q1L))/18014398509481984) + (7514214926474921*sin(q2L)*((1888752292310023*cos(q1L))/18014398509481984 - (5148155107303929*sin(q1L))/9007199254740992))/36893488147419103232))/1152921504606846976 + (9007199067919185*sin(q3L)*((16506520352940097956833727997725*sin(q2L))/20282409603651670423947251286016 - cos(q2L)*((5148155107303929*cos(q1L))/9007199254740992 + (1888752292310023*sin(q1L))/18014398509481984) + (7514214926474921*sin(q2L)*((1888752292310023*cos(q1L))/18014398509481984 - (5148155107303929*sin(q1L))/9007199254740992))/36893488147419103232))/9007199254740992 + 162162510993777435611894002759555259653680159872115681607894875/115792089237316195423570985008687907853269984665640564039457584007913129639936))/9007199254740992 - (7514214926474921*cos(q5L)*(((4503599440548691*cos(q4L))/4503599627370496 - (7514214926474921*sin(q4L))/36893488147419103232)*((9007199067919185*sin(q3L)*((46370457884011341126541404977865*sin(q1L))/81129638414606681695789005144064 - (17012367886825063216155529491255*cos(q1L))/162259276829213363391578010288128 + 13770489658876653055167369550485/83076749736557242056487941267521536))/9007199254740992 - (7514214926474921*sin(q3L)*((16506520352940097956833727997725*cos(q2L))/20282409603651670423947251286016 + (7514214926474921*cos(q2L)*((1888752292310023*cos(q1L))/18014398509481984 - (5148155107303929*sin(q1L))/9007199254740992))/36893488147419103232 + sin(q2L)*((5148155107303929*cos(q1L))/9007199254740992 + (1888752292310023*sin(q1L))/18014398509481984)))/36893488147419103232 + cos(q3L)*((16506520352940097956833727997725*sin(q2L))/20282409603651670423947251286016 - cos(q2L)*((5148155107303929*cos(q1L))/9007199254740992 + (1888752292310023*sin(q1L))/18014398509481984) + (7514214926474921*sin(q2L)*((1888752292310023*cos(q1L))/18014398509481984 - (5148155107303929*sin(q1L))/9007199254740992))/36893488147419103232)) + ((234819211581865*cos(q4L))/1152921504606846976 + (9007199067919185*sin(q4L))/9007199254740992)*((148677514737591106934298605035692608392163854125*cos(q2L))/182687704666362864775460604089535377456991567872 - (127834588709863499538908289888301307693646315855*cos(q1L))/5986310706507378352962293074805895248510699696029696 + (348437586779514700475067630180842053206482623665*sin(q1L))/2993155353253689176481146537402947624255349848014848 + (67682029681889335677290557259385*cos(q2L)*((1888752292310023*cos(q1L))/18014398509481984 - (5148155107303929*sin(q1L))/9007199254740992))/332306998946228968225951765070086144 + (9007199067919185*sin(q2L)*((5148155107303929*cos(q1L))/9007199254740992 + (1888752292310023*sin(q1L))/18014398509481984))/9007199254740992 + 103474418939599489499345508650025439853395886685/3064991081731777716716694054300618367237478244367204352) - (7514214926474921*cos(q4L)*((7514214926474921*cos(q3L)*((16506520352940097956833727997725*cos(q2L))/20282409603651670423947251286016 + (7514214926474921*cos(q2L)*((1888752292310023*cos(q1L))/18014398509481984 - (5148155107303929*sin(q1L))/9007199254740992))/36893488147419103232 + sin(q2L)*((5148155107303929*cos(q1L))/9007199254740992 + (1888752292310023*sin(q1L))/18014398509481984)))/36893488147419103232 - (9007199067919185*cos(q3L)*((46370457884011341126541404977865*sin(q1L))/81129638414606681695789005144064 - (17012367886825063216155529491255*cos(q1L))/162259276829213363391578010288128 + 13770489658876653055167369550485/83076749736557242056487941267521536))/9007199254740992 + sin(q3L)*((16506520352940097956833727997725*sin(q2L))/20282409603651670423947251286016 - cos(q2L)*((5148155107303929*cos(q1L))/9007199254740992 + (1888752292310023*sin(q1L))/18014398509481984) + (7514214926474921*sin(q2L)*((1888752292310023*cos(q1L))/18014398509481984 - (5148155107303929*sin(q1L))/9007199254740992))/36893488147419103232)))/36893488147419103232))/36893488147419103232 + sin(q5L)*(((9007199067919185*cos(q4L))/9007199254740992 - (234819211581865*sin(q4L))/1152921504606846976)*((148677514737591106934298605035692608392163854125*cos(q2L))/182687704666362864775460604089535377456991567872 - (127834588709863499538908289888301307693646315855*cos(q1L))/5986310706507378352962293074805895248510699696029696 + (348437586779514700475067630180842053206482623665*sin(q1L))/2993155353253689176481146537402947624255349848014848 + (67682029681889335677290557259385*cos(q2L)*((1888752292310023*cos(q1L))/18014398509481984 - (5148155107303929*sin(q1L))/9007199254740992))/332306998946228968225951765070086144 + (9007199067919185*sin(q2L)*((5148155107303929*cos(q1L))/9007199254740992 + (1888752292310023*sin(q1L))/18014398509481984))/9007199254740992 + 103474418939599489499345508650025439853395886685/3064991081731777716716694054300618367237478244367204352) - ((7514214926474921*cos(q4L))/36893488147419103232 + (4503599440548691*sin(q4L))/4503599627370496)*((9007199067919185*sin(q3L)*((46370457884011341126541404977865*sin(q1L))/81129638414606681695789005144064 - (17012367886825063216155529491255*cos(q1L))/162259276829213363391578010288128 + 13770489658876653055167369550485/83076749736557242056487941267521536))/9007199254740992 - (7514214926474921*sin(q3L)*((16506520352940097956833727997725*cos(q2L))/20282409603651670423947251286016 + (7514214926474921*cos(q2L)*((1888752292310023*cos(q1L))/18014398509481984 - (5148155107303929*sin(q1L))/9007199254740992))/36893488147419103232 + sin(q2L)*((5148155107303929*cos(q1L))/9007199254740992 + (1888752292310023*sin(q1L))/18014398509481984)))/36893488147419103232 + cos(q3L)*((16506520352940097956833727997725*sin(q2L))/20282409603651670423947251286016 - cos(q2L)*((5148155107303929*cos(q1L))/9007199254740992 + (1888752292310023*sin(q1L))/18014398509481984) + (7514214926474921*sin(q2L)*((1888752292310023*cos(q1L))/18014398509481984 - (5148155107303929*sin(q1L))/9007199254740992))/36893488147419103232)) + (7514214926474921*sin(q4L)*((7514214926474921*cos(q3L)*((16506520352940097956833727997725*cos(q2L))/20282409603651670423947251286016 + (7514214926474921*cos(q2L)*((1888752292310023*cos(q1L))/18014398509481984 - (5148155107303929*sin(q1L))/9007199254740992))/36893488147419103232 + sin(q2L)*((5148155107303929*cos(q1L))/9007199254740992 + (1888752292310023*sin(q1L))/18014398509481984)))/36893488147419103232 - (9007199067919185*cos(q3L)*((46370457884011341126541404977865*sin(q1L))/81129638414606681695789005144064 - (17012367886825063216155529491255*cos(q1L))/162259276829213363391578010288128 + 13770489658876653055167369550485/83076749736557242056487941267521536))/9007199254740992 + sin(q3L)*((16506520352940097956833727997725*sin(q2L))/20282409603651670423947251286016 - cos(q2L)*((5148155107303929*cos(q1L))/9007199254740992 + (1888752292310023*sin(q1L))/18014398509481984) + (7514214926474921*sin(q2L)*((1888752292310023*cos(q1L))/18014398509481984 - (5148155107303929*sin(q1L))/9007199254740992))/36893488147419103232)))/36893488147419103232)))/9007199254740992000 + (202883803014822867*sin(q6L)*((7514214926474921*sin(q5L)*(((4503599440548691*cos(q4L))/4503599627370496 - (7514214926474921*sin(q4L))/36893488147419103232)*((9007199067919185*sin(q3L)*((46370457884011341126541404977865*sin(q1L))/81129638414606681695789005144064 - (17012367886825063216155529491255*cos(q1L))/162259276829213363391578010288128 + 13770489658876653055167369550485/83076749736557242056487941267521536))/9007199254740992 - (7514214926474921*sin(q3L)*((16506520352940097956833727997725*cos(q2L))/20282409603651670423947251286016 + (7514214926474921*cos(q2L)*((1888752292310023*cos(q1L))/18014398509481984 - (5148155107303929*sin(q1L))/9007199254740992))/36893488147419103232 + sin(q2L)*((5148155107303929*cos(q1L))/9007199254740992 + (1888752292310023*sin(q1L))/18014398509481984)))/36893488147419103232 + cos(q3L)*((16506520352940097956833727997725*sin(q2L))/20282409603651670423947251286016 - cos(q2L)*((5148155107303929*cos(q1L))/9007199254740992 + (1888752292310023*sin(q1L))/18014398509481984) + (7514214926474921*sin(q2L)*((1888752292310023*cos(q1L))/18014398509481984 - (5148155107303929*sin(q1L))/9007199254740992))/36893488147419103232)) + ((234819211581865*cos(q4L))/1152921504606846976 + (9007199067919185*sin(q4L))/9007199254740992)*((148677514737591106934298605035692608392163854125*cos(q2L))/182687704666362864775460604089535377456991567872 - (127834588709863499538908289888301307693646315855*cos(q1L))/5986310706507378352962293074805895248510699696029696 + (348437586779514700475067630180842053206482623665*sin(q1L))/2993155353253689176481146537402947624255349848014848 + (67682029681889335677290557259385*cos(q2L)*((1888752292310023*cos(q1L))/18014398509481984 - (5148155107303929*sin(q1L))/9007199254740992))/332306998946228968225951765070086144 + (9007199067919185*sin(q2L)*((5148155107303929*cos(q1L))/9007199254740992 + (1888752292310023*sin(q1L))/18014398509481984))/9007199254740992 + 103474418939599489499345508650025439853395886685/3064991081731777716716694054300618367237478244367204352) - (7514214926474921*cos(q4L)*((7514214926474921*cos(q3L)*((16506520352940097956833727997725*cos(q2L))/20282409603651670423947251286016 + (7514214926474921*cos(q2L)*((1888752292310023*cos(q1L))/18014398509481984 - (5148155107303929*sin(q1L))/9007199254740992))/36893488147419103232 + sin(q2L)*((5148155107303929*cos(q1L))/9007199254740992 + (1888752292310023*sin(q1L))/18014398509481984)))/36893488147419103232 - (9007199067919185*cos(q3L)*((46370457884011341126541404977865*sin(q1L))/81129638414606681695789005144064 - (17012367886825063216155529491255*cos(q1L))/162259276829213363391578010288128 + 13770489658876653055167369550485/83076749736557242056487941267521536))/9007199254740992 + sin(q3L)*((16506520352940097956833727997725*sin(q2L))/20282409603651670423947251286016 - cos(q2L)*((5148155107303929*cos(q1L))/9007199254740992 + (1888752292310023*sin(q1L))/18014398509481984) + (7514214926474921*sin(q2L)*((1888752292310023*cos(q1L))/18014398509481984 - (5148155107303929*sin(q1L))/9007199254740992))/36893488147419103232)))/36893488147419103232))/36893488147419103232 - (9007199067919185*sin(q5L)*((233003667623740560033643537092505706768317191960312467162596875*cos(q2L))/6901746346790563787434755862277025452451108972170386555162524223799296 - (200339157344278917575443724098432450908090682630030995291449625*cos(q1L))/226156424291633194186662080095093570025917938800079226639565593765455331328 + (546062636309760713610973115066597791006802105742542518556166375*sin(q1L))/113078212145816597093331040047546785012958969400039613319782796882727665664 - (81129635049124235038645691064225*cos(q3L)*((46370457884011341126541404977865*sin(q1L))/81129638414606681695789005144064 - (17012367886825063216155529491255*cos(q1L))/162259276829213363391578010288128 + 13770489658876653055167369550485/83076749736557242056487941267521536))/81129638414606681695789005144064 + (2115063383689692319117831580025*sin(q3L)*((46370457884011341126541404977865*sin(q1L))/81129638414606681695789005144064 - (17012367886825063216155529491255*cos(q1L))/162259276829213363391578010288128 + 13770489658876653055167369550485/83076749736557242056487941267521536))/10384593717069655257060992658440192 + (106069577339469832923929692356850887620017617375*cos(q2L)*((1888752292310023*cos(q1L))/18014398509481984 - (5148155107303929*sin(q1L))/9007199254740992))/12554203470773361527671578846415332832204710888928069025792 + (67682029681889335677290557259385*cos(q3L)*((16506520352940097956833727997725*cos(q2L))/20282409603651670423947251286016 + (7514214926474921*cos(q2L)*((1888752292310023*cos(q1L))/18014398509481984 - (5148155107303929*sin(q1L))/9007199254740992))/36893488147419103232 + sin(q2L)*((5148155107303929*cos(q1L))/9007199254740992 + (1888752292310023*sin(q1L))/18014398509481984)))/332306998946228968225951765070086144 + (14115856197532180673579726082375*sin(q2L)*((5148155107303929*cos(q1L))/9007199254740992 + (1888752292310023*sin(q1L))/18014398509481984))/340282366920938463463374607431768211456 - (1764482024691522628700660907665*sin(q3L)*((16506520352940097956833727997725*cos(q2L))/20282409603651670423947251286016 + (7514214926474921*cos(q2L)*((1888752292310023*cos(q1L))/18014398509481984 - (5148155107303929*sin(q1L))/9007199254740992))/36893488147419103232 + sin(q2L)*((5148155107303929*cos(q1L))/9007199254740992 + (1888752292310023*sin(q1L))/18014398509481984)))/42535295865117307932921825928971026432 + 